simulink model "gm_ZynqBF_2tx_fpga"  (R2018b)
settings: Solver=FixedStepDiscrete  StartTime=0.0  StopTime=10.0  FixedStep=(1/420e3)/128  RelTol=1e-3
undefined symbols (not defined in the file or in its folder): a, b, c
libraries: hdlsllib x873, simulink x349
(part 4 of 40)

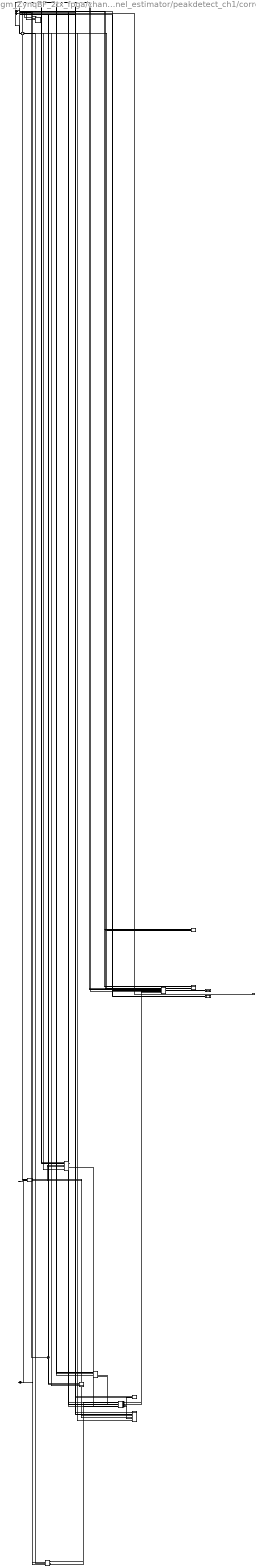
== system gm_ZynqBF_2tx_fpga/channel_estimator/peakdetect_ch1/correlator1 ==
  rx : Inport  OutDataTypeStr=fixdt(1, 16, 15)  PortDimensions=[2]  SampleTime=1.86011904761905e-08
  valid : Inport  Port=2  OutDataTypeStr=boolean  PortDimensions=1  SampleTime=1.86011904761905e-08
  en : Inport  Port=3  OutDataTypeStr=boolean  PortDimensions=1  SampleTime=1.86011904761905e-08
  rst : Inport  Port=4  OutDataTypeStr=boolean  PortDimensions=1  SampleTime=1.86011904761905e-08
  Add : Sum  AccumDataTypeStr=fixdt(1, 36, 16)  OutDataTypeStr=fixdt(1, 32, 16)  SampleTime=1.86011904761905e-08
  Compare To Constant2 : simulink/Logic and Bit Operations/Compare To Constant  relop===  const=fi(0,0,8,0,'hex','02')  OutDataTypeStr=boolean
  Compare To Constant3 : simulink/Logic and Bit Operations/Compare To Constant  relop===  const=fi(0,0,8,0,'hex','01')  OutDataTypeStr=boolean
  Constant : Constant  Value=[0;1;2;3;4;5;6;7;8;9;10;11;12;13;14;15;16;17;18;19;20;21;22;23;24;25;26;27;28;29;30;31;32;33;34;35;36;37;38;39;40;41;42;43;44;45;46;47;48;49;50;51;52;53;54;55;56;57;58;59;60;61;62;63]  OutDataTypeStr=fixdt(0, 6, 0)  SampleTime=-1
  Delay{1,4..8} (6 alike) : Delay  DelayLength=double(1)  InitialCondition=0  InputProcessing=Inherited  SampleTime=1.86011904761905e-08
  Delay2 : Delay  DelayLength=double(2)  InitialCondition=0  InputProcessing=Inherited  SampleTime=1.86011904761905e-08
  Delay3 : Delay  DelayLength=double(4)  InitialCondition=0  InputProcessing=Inherited  SampleTime=1.86011904761905e-08
  HDL Counter1 : hdlsllib/Sources/HDL Counter  CountType=Count limited  CountInit=double(0)  CountStep=double(1)  CountMax=double(2)  CountFromType=Initial value  CountFrom=double(0)  CountResetPort=off  CountLoadPort=off  CountEnbPort=on  CountDirPort=off  CountDataType=Unsigned  CountWordLen=8  CountFracLen=0  CountSampTime=1.86011904761905e-08
      settings: SourceProductBaseCode=HD
  Logical Operator : Logic  Operator=OR  Inputs=1  AllPortsSameDT=off  OutDataTypeStr=boolean  SampleTime=1.86011904761905e-08
  Logical Operator10 : Logic  AllPortsSameDT=off  OutDataTypeStr=boolean  SampleTime=1.86011904761905e-08
  Logical Operator4 : Logic  Inputs=1  AllPortsSameDT=off  OutDataTypeStr=boolean  SampleTime=1.86011904761905e-08
  Logical Operator5 : Logic  Inputs=1  AllPortsSameDT=off  OutDataTypeStr=boolean  SampleTime=1.86011904761905e-08
  Logical Operator6 : Logic  AllPortsSameDT=off  OutDataTypeStr=boolean  SampleTime=1.86011904761905e-08
  Logical Operator8 : Logic  AllPortsSameDT=off  OutDataTypeStr=boolean  SampleTime=1.86011904761905e-08
  Logical Operator9 : Logic  Operator=OR  Inputs=3  AllPortsSameDT=off  OutDataTypeStr=boolean  SampleTime=1.86011904761905e-08
  Sum of Elements1 : Sum  Inputs=+  AccumDataTypeStr=fixdt(1, 35, 16)  OutDataTypeStr=fixdt(1, 35, 16)  SampleTime=1.86011904761905e-08
  Sum of Elements2 : Sum  Inputs=+  AccumDataTypeStr=fixdt(1, 35, 16)  OutDataTypeStr=fixdt(1, 35, 16)  SampleTime=1.86011904761905e-08
  all_u : Subsystem
  all_u1 : Subsystem
  correlation_config : Subsystem
  correlator_en : Subsystem
  correlator_i_instance1 : Subsystem
  correlator_i_instance10 : Subsystem
  correlator_i_instance11 : Subsystem
  correlator_i_instance12 : Subsystem
  correlator_i_instance13 : Subsystem
  correlator_i_instance14 : Subsystem
  correlator_i_instance15 : Subsystem
  correlator_i_instance16 : Subsystem
  correlator_i_instance17 : Subsystem
  correlator_i_instance18 : Subsystem
  correlator_i_instance19 : Subsystem
  correlator_i_instance2 : Subsystem
  correlator_i_instance20 : Subsystem
  correlator_i_instance21 : Subsystem
  correlator_i_instance22 : Subsystem
  correlator_i_instance23 : Subsystem
  correlator_i_instance24 : Subsystem
  correlator_i_instance25 : Subsystem
  correlator_i_instance26 : Subsystem
  correlator_i_instance27 : Subsystem
  correlator_i_instance28 : Subsystem
  correlator_i_instance29 : Subsystem
  correlator_i_instance3 : Subsystem
  correlator_i_instance30 : Subsystem
  correlator_i_instance31 : Subsystem
  correlator_i_instance32 : Subsystem
  correlator_i_instance33 : Subsystem
  correlator_i_instance34 : Subsystem
  correlator_i_instance35 : Subsystem
  correlator_i_instance36 : Subsystem
  correlator_i_instance37 : Subsystem
  correlator_i_instance38 : Subsystem
  correlator_i_instance39 : Subsystem
  correlator_i_instance4 : Subsystem
  correlator_i_instance40 : Subsystem
  correlator_i_instance41 : Subsystem
  correlator_i_instance42 : Subsystem
  correlator_i_instance43 : Subsystem
  correlator_i_instance44 : Subsystem
  correlator_i_instance45 : Subsystem
  correlator_i_instance46 : Subsystem
  correlator_i_instance47 : Subsystem
  correlator_i_instance48 : Subsystem
  correlator_i_instance49 : Subsystem
  correlator_i_instance5 : Subsystem
  correlator_i_instance50 : Subsystem
  correlator_i_instance51 : Subsystem
  correlator_i_instance52 : Subsystem
  correlator_i_instance53 : Subsystem
  correlator_i_instance54 : Subsystem
  correlator_i_instance55 : Subsystem
  correlator_i_instance56 : Subsystem
  correlator_i_instance57 : Subsystem
  correlator_i_instance58 : Subsystem
  correlator_i_instance59 : Subsystem
  correlator_i_instance6 : Subsystem
  correlator_i_instance60 : Subsystem
  correlator_i_instance61 : Subsystem
  correlator_i_instance62 : Subsystem
  correlator_i_instance63 : Subsystem
  correlator_i_instance64 : Subsystem
  correlator_i_instance7 : Subsystem
  correlator_i_instance8 : Subsystem
  correlator_i_instance9 : Subsystem
  correlator_q_instance1 : Subsystem
  correlator_q_instance10 : Subsystem
  correlator_q_instance11 : Subsystem
  correlator_q_instance12 : Subsystem
  correlator_q_instance13 : Subsystem
  correlator_q_instance14 : Subsystem
  correlator_q_instance15 : Subsystem
  correlator_q_instance16 : Subsystem
  correlator_q_instance17 : Subsystem
  correlator_q_instance18 : Subsystem
  correlator_q_instance19 : Subsystem
  correlator_q_instance2 : Subsystem
  correlator_q_instance20 : Subsystem
  correlator_q_instance21 : Subsystem
  correlator_q_instance22 : Subsystem
  correlator_q_instance23 : Subsystem
  correlator_q_instance24 : Subsystem
  correlator_q_instance25 : Subsystem
  correlator_q_instance26 : Subsystem
  correlator_q_instance27 : Subsystem
  correlator_q_instance28 : Subsystem
  correlator_q_instance29 : Subsystem
  correlator_q_instance3 : Subsystem
  correlator_q_instance30 : Subsystem
  correlator_q_instance31 : Subsystem
  correlator_q_instance32 : Subsystem
  correlator_q_instance33 : Subsystem
  correlator_q_instance34 : Subsystem
  correlator_q_instance35 : Subsystem
  correlator_q_instance36 : Subsystem
  correlator_q_instance37 : Subsystem
  correlator_q_instance38 : Subsystem
  correlator_q_instance39 : Subsystem
  correlator_q_instance4 : Subsystem
  correlator_q_instance40 : Subsystem
  correlator_q_instance41 : Subsystem
  correlator_q_instance42 : Subsystem
  correlator_q_instance43 : Subsystem
  correlator_q_instance44 : Subsystem
  correlator_q_instance45 : Subsystem
  correlator_q_instance46 : Subsystem
  correlator_q_instance47 : Subsystem
  correlator_q_instance48 : Subsystem
  correlator_q_instance49 : Subsystem
  correlator_q_instance5 : Subsystem
  correlator_q_instance50 : Subsystem
  correlator_q_instance51 : Subsystem
  correlator_q_instance52 : Subsystem
  correlator_q_instance53 : Subsystem
  correlator_q_instance54 : Subsystem
  correlator_q_instance55 : Subsystem
  correlator_q_instance56 : Subsystem
  correlator_q_instance57 : Subsystem
  correlator_q_instance58 : Subsystem
  correlator_q_instance59 : Subsystem
  correlator_q_instance6 : Subsystem
  correlator_q_instance60 : Subsystem
  correlator_q_instance61 : Subsystem
  correlator_q_instance62 : Subsystem
  correlator_q_instance63 : Subsystem
  correlator_q_instance64 : Subsystem
  correlator_q_instance7 : Subsystem
  correlator_q_instance8 : Subsystem
  correlator_q_instance9 : Subsystem
  data_in : Subsystem
  gold_sequences : Subsystem
  rx_ram_i_instance1 : Subsystem
  rx_ram_i_instance10 : Subsystem
  rx_ram_i_instance11 : Subsystem
  rx_ram_i_instance12 : Subsystem
  rx_ram_i_instance13 : Subsystem
  rx_ram_i_instance14 : Subsystem
  rx_ram_i_instance15 : Subsystem
  rx_ram_i_instance16 : Subsystem
  rx_ram_i_instance17 : Subsystem
  rx_ram_i_instance18 : Subsystem
  rx_ram_i_instance19 : Subsystem
  rx_ram_i_instance2 : Subsystem
  rx_ram_i_instance20 : Subsystem
  rx_ram_i_instance21 : Subsystem
  rx_ram_i_instance22 : Subsystem
  rx_ram_i_instance23 : Subsystem
  rx_ram_i_instance24 : Subsystem
  rx_ram_i_instance25 : Subsystem
  rx_ram_i_instance26 : Subsystem
  rx_ram_i_instance27 : Subsystem
  rx_ram_i_instance28 : Subsystem
  rx_ram_i_instance29 : Subsystem
  rx_ram_i_instance3 : Subsystem
  rx_ram_i_instance30 : Subsystem
  rx_ram_i_instance31 : Subsystem
  rx_ram_i_instance32 : Subsystem
  rx_ram_i_instance33 : Subsystem
  rx_ram_i_instance34 : Subsystem
  rx_ram_i_instance35 : Subsystem
  rx_ram_i_instance36 : Subsystem
  rx_ram_i_instance37 : Subsystem
  rx_ram_i_instance38 : Subsystem
  rx_ram_i_instance39 : Subsystem
  rx_ram_i_instance4 : Subsystem
  rx_ram_i_instance40 : Subsystem
  rx_ram_i_instance41 : Subsystem
  rx_ram_i_instance42 : Subsystem
  rx_ram_i_instance43 : Subsystem
  rx_ram_i_instance44 : Subsystem
  rx_ram_i_instance45 : Subsystem
  rx_ram_i_instance46 : Subsystem
  rx_ram_i_instance47 : Subsystem
  rx_ram_i_instance48 : Subsystem
  rx_ram_i_instance49 : Subsystem
  rx_ram_i_instance5 : Subsystem
  rx_ram_i_instance50 : Subsystem
  rx_ram_i_instance51 : Subsystem
  rx_ram_i_instance52 : Subsystem
  rx_ram_i_instance53 : Subsystem
  rx_ram_i_instance54 : Subsystem
  rx_ram_i_instance55 : Subsystem
  rx_ram_i_instance56 : Subsystem
  rx_ram_i_instance57 : Subsystem
  rx_ram_i_instance58 : Subsystem
  rx_ram_i_instance59 : Subsystem
  rx_ram_i_instance6 : Subsystem
  rx_ram_i_instance60 : Subsystem
  rx_ram_i_instance61 : Subsystem
  rx_ram_i_instance62 : Subsystem
  rx_ram_i_instance63 : Subsystem
  rx_ram_i_instance64 : Subsystem
  rx_ram_i_instance7 : Subsystem
  rx_ram_i_instance8 : Subsystem
  rx_ram_i_instance9 : Subsystem
  rx_ram_q_instance1 : Subsystem
  rx_ram_q_instance10 : Subsystem
  rx_ram_q_instance11 : Subsystem
  rx_ram_q_instance12 : Subsystem
  rx_ram_q_instance13 : Subsystem
  rx_ram_q_instance14 : Subsystem
  rx_ram_q_instance15 : Subsystem
  rx_ram_q_instance16 : Subsystem
  rx_ram_q_instance17 : Subsystem
  rx_ram_q_instance18 : Subsystem
  rx_ram_q_instance19 : Subsystem
  rx_ram_q_instance2 : Subsystem
  rx_ram_q_instance20 : Subsystem
  rx_ram_q_instance21 : Subsystem
  rx_ram_q_instance22 : Subsystem
  rx_ram_q_instance23 : Subsystem
  rx_ram_q_instance24 : Subsystem
  rx_ram_q_instance25 : Subsystem
  rx_ram_q_instance26 : Subsystem
  rx_ram_q_instance27 : Subsystem
  rx_ram_q_instance28 : Subsystem
  rx_ram_q_instance29 : Subsystem
  rx_ram_q_instance3 : Subsystem
  rx_ram_q_instance30 : Subsystem
  rx_ram_q_instance31 : Subsystem
  rx_ram_q_instance32 : Subsystem
  rx_ram_q_instance33 : Subsystem
  rx_ram_q_instance34 : Subsystem
  rx_ram_q_instance35 : Subsystem
  rx_ram_q_instance36 : Subsystem
  rx_ram_q_instance37 : Subsystem
  rx_ram_q_instance38 : Subsystem
  rx_ram_q_instance39 : Subsystem
  rx_ram_q_instance4 : Subsystem
  rx_ram_q_instance40 : Subsystem
  rx_ram_q_instance41 : Subsystem
  rx_ram_q_instance42 : Subsystem
  rx_ram_q_instance43 : Subsystem
  rx_ram_q_instance44 : Subsystem
  rx_ram_q_instance45 : Subsystem
  rx_ram_q_instance46 : Subsystem
  rx_ram_q_instance47 : Subsystem
  rx_ram_q_instance48 : Subsystem
  rx_ram_q_instance49 : Subsystem
  rx_ram_q_instance5 : Subsystem
  rx_ram_q_instance50 : Subsystem
  rx_ram_q_instance51 : Subsystem
  rx_ram_q_instance52 : Subsystem
  rx_ram_q_instance53 : Subsystem
  rx_ram_q_instance54 : Subsystem
  rx_ram_q_instance55 : Subsystem
  rx_ram_q_instance56 : Subsystem
  rx_ram_q_instance57 : Subsystem
  rx_ram_q_instance58 : Subsystem
  rx_ram_q_instance59 : Subsystem
  rx_ram_q_instance6 : Subsystem
  rx_ram_q_instance60 : Subsystem
  rx_ram_q_instance61 : Subsystem
  rx_ram_q_instance62 : Subsystem
  rx_ram_q_instance63 : Subsystem
  rx_ram_q_instance64 : Subsystem
  rx_ram_q_instance7 : Subsystem
  rx_ram_q_instance8 : Subsystem
  rx_ram_q_instance9 : Subsystem
  select_rx_i : Selector  IndexMode=Zero-based  SampleTime=1.86011904761905e-08  IndexOptions=Index vector (dialog)  Indices=double(0)  OutputSizes=double(1)
  select_rx_q : Selector  IndexMode=Zero-based  SampleTime=1.86011904761905e-08  IndexOptions=Index vector (dialog)  Indices=double(1)  OutputSizes=double(1)
  shift_rx : Subsystem
  shift_rx1 : Subsystem
  sum_elements_i_instance1 : Subsystem
  sum_elements_i_instance2 : Subsystem
  sum_elements_i_instance3 : Subsystem
  sum_elements_i_instance4 : Subsystem
  sum_elements_i_instance5 : Subsystem
  sum_elements_i_instance6 : Subsystem
  sum_elements_i_instance7 : Subsystem
  sum_elements_i_instance8 : Subsystem
  sum_elements_q_instance1 : Subsystem
  sum_elements_q_instance2 : Subsystem
  sum_elements_q_instance3 : Subsystem
  sum_elements_q_instance4 : Subsystem
  sum_elements_q_instance5 : Subsystem
  sum_elements_q_instance6 : Subsystem
  sum_elements_q_instance7 : Subsystem
  sum_elements_q_instance8 : Subsystem
  t{,1,4..5,8,10} (6 alike) : Demux  Outputs=64
  t{2..3,6..7,9,11} (6 alike) : Mux  Inputs=64
  t12 : Demux  Outputs=8
  t{13..14,16..17} (4 alike) : Mux  Inputs=8
  t15 : Demux  Outputs=8
  dout : Outport
  dval : Outport  Port=2
  step : Outport  Port=3
  wires:
  rx/1 -> select_rx_q/1, select_rx_i/1
  valid/1 -> data_in/2(valid)
  en/1 -> Logical Operator10/2
  rst/1 -> correlation_config/1(rst), data_in/1(rst)
  Add/1 -> Delay7/1
  Compare To Constant2/1 -> Logical Operator9/3, step/1
  Compare To Constant3/1 -> Logical Operator10/1
  Constant/1 -> t10/1, t8/1
  Delay1/1 -> Add/1
  Delay2/1 -> sum_elements_q_instance8/2(start), sum_elements_q_instance7/2(start), sum_elements_q_instance6/2(start), sum_elements_q_instance5/2(start), sum_elements_q_instance4/2(start), sum_elements_q_instance3/2(start), sum_elements_q_instance2/2(start), sum_elements_i_instance8/2(start), sum_elements_i_instance7/2(start), sum_elements_i_instance6/2(start), sum_elements_i_instance5/2(start), sum_elements_i_instance4/2(start), sum_elements_i_instance3/2(start), sum_elements_i_instance2/2(start), sum_elements_i_instance1/2(start), sum_elements_q_instance1/2(start)
  Delay3/1 -> Logical Operator9/2, dval/1
  Delay4/1 -> Delay8/1, Delay6/1, rx_ram_q_instance64/6(shift), rx_ram_q_instance63/6(shift), rx_ram_q_instance62/6(shift), rx_ram_q_instance61/6(shift), rx_ram_q_instance60/6(shift), rx_ram_q_instance59/6(shift), rx_ram_q_instance58/6(shift), rx_ram_q_instance57/6(shift), rx_ram_q_instance56/6(shift), rx_ram_q_instance55/6(shift), rx_ram_q_instance54/6(shift), rx_ram_q_instance53/6(shift), rx_ram_q_instance52/6(shift), rx_ram_q_instance51/6(shift), rx_ram_q_instance50/6(shift), rx_ram_q_instance49/6(shift), rx_ram_q_instance48/6(shift), rx_ram_q_instance47/6(shift), rx_ram_q_instance46/6(shift), rx_ram_q_instance45/6(shift), rx_ram_q_instance44/6(shift), rx_ram_q_instance43/6(shift), rx_ram_q_instance42/6(shift), rx_ram_q_instance41/6(shift), rx_ram_q_instance40/6(shift), rx_ram_q_instance39/6(shift), rx_ram_q_instance38/6(shift), rx_ram_q_instance37/6(shift), rx_ram_q_instance36/6(shift), rx_ram_q_instance35/6(shift), rx_ram_q_instance34/6(shift), rx_ram_q_instance33/6(shift), rx_ram_q_instance32/6(shift), rx_ram_q_instance31/6(shift), rx_ram_q_instance30/6(shift), rx_ram_q_instance29/6(shift), rx_ram_q_instance28/6(shift), rx_ram_q_instance27/6(shift), rx_ram_q_instance26/6(shift), rx_ram_q_instance25/6(shift), rx_ram_q_instance24/6(shift), rx_ram_q_instance23/6(shift), rx_ram_q_instance22/6(shift), rx_ram_q_instance21/6(shift), rx_ram_q_instance20/6(shift), rx_ram_q_instance19/6(shift), rx_ram_q_instance18/6(shift), rx_ram_q_instance17/6(shift), rx_ram_q_instance16/6(shift), rx_ram_q_instance15/6(shift), rx_ram_q_instance14/6(shift), rx_ram_q_instance13/6(shift), rx_ram_q_instance12/6(shift), rx_ram_q_instance11/6(shift), rx_ram_q_instance10/6(shift), rx_ram_q_instance9/6(shift), rx_ram_q_instance8/6(shift), rx_ram_q_instance7/6(shift), rx_ram_q_instance6/6(shift), rx_ram_q_instance5/6(shift), rx_ram_q_instance4/6(shift), rx_ram_q_instance3/6(shift), rx_ram_q_instance2/6(shift), rx_ram_i_instance64/6(shift), rx_ram_i_instance63/6(shift), rx_ram_i_instance62/6(shift), rx_ram_i_instance61/6(shift), rx_ram_i_instance60/6(shift), rx_ram_i_instance59/6(shift), rx_ram_i_instance58/6(shift), rx_ram_i_instance57/6(shift), rx_ram_i_instance56/6(shift), rx_ram_i_instance55/6(shift), rx_ram_i_instance54/6(shift), rx_ram_i_instance53/6(shift), rx_ram_i_instance52/6(shift), rx_ram_i_instance51/6(shift), rx_ram_i_instance50/6(shift), rx_ram_i_instance49/6(shift), rx_ram_i_instance48/6(shift), rx_ram_i_instance47/6(shift), rx_ram_i_instance46/6(shift), rx_ram_i_instance45/6(shift), rx_ram_i_instance44/6(shift), rx_ram_i_instance43/6(shift), rx_ram_i_instance42/6(shift), rx_ram_i_instance41/6(shift), rx_ram_i_instance40/6(shift), rx_ram_i_instance39/6(shift), rx_ram_i_instance38/6(shift), rx_ram_i_instance37/6(shift), rx_ram_i_instance36/6(shift), rx_ram_i_instance35/6(shift), rx_ram_i_instance34/6(shift), rx_ram_i_instance33/6(shift), rx_ram_i_instance32/6(shift), rx_ram_i_instance31/6(shift), rx_ram_i_instance30/6(shift), rx_ram_i_instance29/6(shift), rx_ram_i_instance28/6(shift), rx_ram_i_instance27/6(shift), rx_ram_i_instance26/6(shift), rx_ram_i_instance25/6(shift), rx_ram_i_instance24/6(shift), rx_ram_i_instance23/6(shift), rx_ram_i_instance22/6(shift), rx_ram_i_instance21/6(shift), rx_ram_i_instance20/6(shift), rx_ram_i_instance19/6(shift), rx_ram_i_instance18/6(shift), rx_ram_i_instance17/6(shift), rx_ram_i_instance16/6(shift), rx_ram_i_instance15/6(shift), rx_ram_i_instance14/6(shift), rx_ram_i_instance13/6(shift), rx_ram_i_instance12/6(shift), rx_ram_i_instance11/6(shift), rx_ram_i_instance10/6(shift), rx_ram_i_instance9/6(shift), rx_ram_i_instance8/6(shift), rx_ram_i_instance7/6(shift), rx_ram_i_instance6/6(shift), rx_ram_i_instance5/6(shift), rx_ram_i_instance4/6(shift), rx_ram_i_instance3/6(shift), rx_ram_i_instance2/6(shift), rx_ram_i_instance1/6(shift), rx_ram_q_instance1/6(shift)
  Delay5/1 -> Add/2
  Delay6/1 -> shift_rx/2(shift)
  Delay7/1 -> dout/1
  Delay8/1 -> shift_rx1/2(shift)
  HDL Counter1/1 -> Compare To Constant3/1, Compare To Constant2/1
  Logical Operator/1 -> correlation_config/2(vin)
  Logical Operator10/1 -> Logical Operator9/1
  Logical Operator4/1 -> Logical Operator6/1
  Logical Operator5/1 -> Logical Operator6/2
  Logical Operator6/1 -> Delay2/1, correlator_en/2(done)
  Logical Operator8/1 -> Delay3/1
  Logical Operator9/1 -> HDL Counter1/1
  Sum of Elements1/1 -> Delay1/1
  Sum of Elements2/1 -> Delay5/1
  all_u/1(y) -> Logical Operator8/1
  all_u1/1(y) -> Logical Operator8/2
  correlation_config/1(addr) -> correlator_en/3(addri)
  correlation_config/2(shift) -> Delay4/1
  correlation_config/3(vout) -> correlator_en/1(valid)
  correlator_en/1(start) -> correlator_q_instance64/3(start), correlator_q_instance63/3(start), correlator_q_instance62/3(start), correlator_q_instance61/3(start), correlator_q_instance60/3(start), correlator_q_instance59/3(start), correlator_q_instance58/3(start), correlator_q_instance57/3(start), correlator_q_instance56/3(start), correlator_q_instance55/3(start), correlator_q_instance54/3(start), correlator_q_instance53/3(start), correlator_q_instance52/3(start), correlator_q_instance51/3(start), correlator_q_instance50/3(start), correlator_q_instance49/3(start), correlator_q_instance48/3(start), correlator_q_instance47/3(start), correlator_q_instance46/3(start), correlator_q_instance45/3(start), correlator_q_instance44/3(start), correlator_q_instance43/3(start), correlator_q_instance42/3(start), correlator_q_instance41/3(start), correlator_q_instance40/3(start), correlator_q_instance39/3(start), correlator_q_instance38/3(start), correlator_q_instance37/3(start), correlator_q_instance36/3(start), correlator_q_instance35/3(start), correlator_q_instance34/3(start), correlator_q_instance33/3(start), correlator_q_instance32/3(start), correlator_q_instance31/3(start), correlator_q_instance30/3(start), correlator_q_instance29/3(start), correlator_q_instance28/3(start), correlator_q_instance27/3(start), correlator_q_instance26/3(start), correlator_q_instance25/3(start), correlator_q_instance24/3(start), correlator_q_instance23/3(start), correlator_q_instance22/3(start), correlator_q_instance21/3(start), correlator_q_instance20/3(start), correlator_q_instance19/3(start), correlator_q_instance18/3(start), correlator_q_instance17/3(start), correlator_q_instance16/3(start), correlator_q_instance15/3(start), correlator_q_instance14/3(start), correlator_q_instance13/3(start), correlator_q_instance12/3(start), correlator_q_instance11/3(start), correlator_q_instance10/3(start), correlator_q_instance9/3(start), correlator_q_instance8/3(start), correlator_q_instance7/3(start), correlator_q_instance6/3(start), correlator_q_instance5/3(start), correlator_q_instance4/3(start), correlator_q_instance3/3(start), correlator_q_instance2/3(start), correlator_i_instance64/3(start), correlator_i_instance63/3(start), correlator_i_instance62/3(start), correlator_i_instance61/3(start), correlator_i_instance60/3(start), correlator_i_instance59/3(start), correlator_i_instance58/3(start), correlator_i_instance57/3(start), correlator_i_instance56/3(start), correlator_i_instance55/3(start), correlator_i_instance54/3(start), correlator_i_instance53/3(start), correlator_i_instance52/3(start), correlator_i_instance51/3(start), correlator_i_instance50/3(start), correlator_i_instance49/3(start), correlator_i_instance48/3(start), correlator_i_instance47/3(start), correlator_i_instance46/3(start), correlator_i_instance45/3(start), correlator_i_instance44/3(start), correlator_i_instance43/3(start), correlator_i_instance42/3(start), correlator_i_instance41/3(start), correlator_i_instance40/3(start), correlator_i_instance39/3(start), correlator_i_instance38/3(start), correlator_i_instance37/3(start), correlator_i_instance36/3(start), correlator_i_instance35/3(start), correlator_i_instance34/3(start), correlator_i_instance33/3(start), correlator_i_instance32/3(start), correlator_i_instance31/3(start), correlator_i_instance30/3(start), correlator_i_instance29/3(start), correlator_i_instance28/3(start), correlator_i_instance27/3(start), correlator_i_instance26/3(start), correlator_i_instance25/3(start), correlator_i_instance24/3(start), correlator_i_instance23/3(start), correlator_i_instance22/3(start), correlator_i_instance21/3(start), correlator_i_instance20/3(start), correlator_i_instance19/3(start), correlator_i_instance18/3(start), correlator_i_instance17/3(start), correlator_i_instance16/3(start), correlator_i_instance15/3(start), correlator_i_instance14/3(start), correlator_i_instance13/3(start), correlator_i_instance12/3(start), correlator_i_instance11/3(start), correlator_i_instance10/3(start), correlator_i_instance9/3(start), correlator_i_instance8/3(start), correlator_i_instance7/3(start), correlator_i_instance6/3(start), correlator_i_instance5/3(start), correlator_i_instance4/3(start), correlator_i_instance3/3(start), correlator_i_instance2/3(start), correlator_q_instance1/3(start), correlator_i_instance1/3(start)
  correlator_en/2(en) -> correlator_q_instance64/4(vin), correlator_q_instance63/4(vin), correlator_q_instance62/4(vin), correlator_q_instance61/4(vin), correlator_q_instance60/4(vin), correlator_q_instance59/4(vin), correlator_q_instance58/4(vin), correlator_q_instance57/4(vin), correlator_q_instance56/4(vin), correlator_q_instance55/4(vin), correlator_q_instance54/4(vin), correlator_q_instance53/4(vin), correlator_q_instance52/4(vin), correlator_q_instance51/4(vin), correlator_q_instance50/4(vin), correlator_q_instance49/4(vin), correlator_q_instance48/4(vin), correlator_q_instance47/4(vin), correlator_q_instance46/4(vin), correlator_q_instance45/4(vin), correlator_q_instance44/4(vin), correlator_q_instance43/4(vin), correlator_q_instance42/4(vin), correlator_q_instance41/4(vin), correlator_q_instance40/4(vin), correlator_q_instance39/4(vin), correlator_q_instance38/4(vin), correlator_q_instance37/4(vin), correlator_q_instance36/4(vin), correlator_q_instance35/4(vin), correlator_q_instance34/4(vin), correlator_q_instance33/4(vin), correlator_q_instance32/4(vin), correlator_q_instance31/4(vin), correlator_q_instance30/4(vin), correlator_q_instance29/4(vin), correlator_q_instance28/4(vin), correlator_q_instance27/4(vin), correlator_q_instance26/4(vin), correlator_q_instance25/4(vin), correlator_q_instance24/4(vin), correlator_q_instance23/4(vin), correlator_q_instance22/4(vin), correlator_q_instance21/4(vin), correlator_q_instance20/4(vin), correlator_q_instance19/4(vin), correlator_q_instance18/4(vin), correlator_q_instance17/4(vin), correlator_q_instance16/4(vin), correlator_q_instance15/4(vin), correlator_q_instance14/4(vin), correlator_q_instance13/4(vin), correlator_q_instance12/4(vin), correlator_q_instance11/4(vin), correlator_q_instance10/4(vin), correlator_q_instance9/4(vin), correlator_q_instance8/4(vin), correlator_q_instance7/4(vin), correlator_q_instance6/4(vin), correlator_q_instance5/4(vin), correlator_q_instance4/4(vin), correlator_q_instance3/4(vin), correlator_q_instance2/4(vin), correlator_i_instance64/4(vin), correlator_i_instance63/4(vin), correlator_i_instance62/4(vin), correlator_i_instance61/4(vin), correlator_i_instance60/4(vin), correlator_i_instance59/4(vin), correlator_i_instance58/4(vin), correlator_i_instance57/4(vin), correlator_i_instance56/4(vin), correlator_i_instance55/4(vin), correlator_i_instance54/4(vin), correlator_i_instance53/4(vin), correlator_i_instance52/4(vin), correlator_i_instance51/4(vin), correlator_i_instance50/4(vin), correlator_i_instance49/4(vin), correlator_i_instance48/4(vin), correlator_i_instance47/4(vin), correlator_i_instance46/4(vin), correlator_i_instance45/4(vin), correlator_i_instance44/4(vin), correlator_i_instance43/4(vin), correlator_i_instance42/4(vin), correlator_i_instance41/4(vin), correlator_i_instance40/4(vin), correlator_i_instance39/4(vin), correlator_i_instance38/4(vin), correlator_i_instance37/4(vin), correlator_i_instance36/4(vin), correlator_i_instance35/4(vin), correlator_i_instance34/4(vin), correlator_i_instance33/4(vin), correlator_i_instance32/4(vin), correlator_i_instance31/4(vin), correlator_i_instance30/4(vin), correlator_i_instance29/4(vin), correlator_i_instance28/4(vin), correlator_i_instance27/4(vin), correlator_i_instance26/4(vin), correlator_i_instance25/4(vin), correlator_i_instance24/4(vin), correlator_i_instance23/4(vin), correlator_i_instance22/4(vin), correlator_i_instance21/4(vin), correlator_i_instance20/4(vin), correlator_i_instance19/4(vin), correlator_i_instance18/4(vin), correlator_i_instance17/4(vin), correlator_i_instance16/4(vin), correlator_i_instance15/4(vin), correlator_i_instance14/4(vin), correlator_i_instance13/4(vin), correlator_i_instance12/4(vin), correlator_i_instance11/4(vin), correlator_i_instance10/4(vin), correlator_i_instance9/4(vin), correlator_i_instance8/4(vin), correlator_i_instance7/4(vin), correlator_i_instance6/4(vin), correlator_i_instance5/4(vin), correlator_i_instance4/4(vin), correlator_i_instance3/4(vin), correlator_i_instance2/4(vin), correlator_q_instance1/4(vin), correlator_i_instance1/4(vin)
  correlator_en/3(gs_addr) -> gold_sequences/1(addr)
  correlator_en/4(rx_addr) -> rx_ram_q_instance64/5(raddr), rx_ram_q_instance63/5(raddr), rx_ram_q_instance62/5(raddr), rx_ram_q_instance61/5(raddr), rx_ram_q_instance60/5(raddr), rx_ram_q_instance59/5(raddr), rx_ram_q_instance58/5(raddr), rx_ram_q_instance57/5(raddr), rx_ram_q_instance56/5(raddr), rx_ram_q_instance55/5(raddr), rx_ram_q_instance54/5(raddr), rx_ram_q_instance53/5(raddr), rx_ram_q_instance52/5(raddr), rx_ram_q_instance51/5(raddr), rx_ram_q_instance50/5(raddr), rx_ram_q_instance49/5(raddr), rx_ram_q_instance48/5(raddr), rx_ram_q_instance47/5(raddr), rx_ram_q_instance46/5(raddr), rx_ram_q_instance45/5(raddr), rx_ram_q_instance44/5(raddr), rx_ram_q_instance43/5(raddr), rx_ram_q_instance42/5(raddr), rx_ram_q_instance41/5(raddr), rx_ram_q_instance40/5(raddr), rx_ram_q_instance39/5(raddr), rx_ram_q_instance38/5(raddr), rx_ram_q_instance37/5(raddr), rx_ram_q_instance36/5(raddr), rx_ram_q_instance35/5(raddr), rx_ram_q_instance34/5(raddr), rx_ram_q_instance33/5(raddr), rx_ram_q_instance32/5(raddr), rx_ram_q_instance31/5(raddr), rx_ram_q_instance30/5(raddr), rx_ram_q_instance29/5(raddr), rx_ram_q_instance28/5(raddr), rx_ram_q_instance27/5(raddr), rx_ram_q_instance26/5(raddr), rx_ram_q_instance25/5(raddr), rx_ram_q_instance24/5(raddr), rx_ram_q_instance23/5(raddr), rx_ram_q_instance22/5(raddr), rx_ram_q_instance21/5(raddr), rx_ram_q_instance20/5(raddr), rx_ram_q_instance19/5(raddr), rx_ram_q_instance18/5(raddr), rx_ram_q_instance17/5(raddr), rx_ram_q_instance16/5(raddr), rx_ram_q_instance15/5(raddr), rx_ram_q_instance14/5(raddr), rx_ram_q_instance13/5(raddr), rx_ram_q_instance12/5(raddr), rx_ram_q_instance11/5(raddr), rx_ram_q_instance10/5(raddr), rx_ram_q_instance9/5(raddr), rx_ram_q_instance8/5(raddr), rx_ram_q_instance7/5(raddr), rx_ram_q_instance6/5(raddr), rx_ram_q_instance5/5(raddr), rx_ram_q_instance4/5(raddr), rx_ram_q_instance3/5(raddr), rx_ram_q_instance2/5(raddr), rx_ram_i_instance64/5(raddr), rx_ram_i_instance63/5(raddr), rx_ram_i_instance62/5(raddr), rx_ram_i_instance61/5(raddr), rx_ram_i_instance60/5(raddr), rx_ram_i_instance59/5(raddr), rx_ram_i_instance58/5(raddr), rx_ram_i_instance57/5(raddr), rx_ram_i_instance56/5(raddr), rx_ram_i_instance55/5(raddr), rx_ram_i_instance54/5(raddr), rx_ram_i_instance53/5(raddr), rx_ram_i_instance52/5(raddr), rx_ram_i_instance51/5(raddr), rx_ram_i_instance50/5(raddr), rx_ram_i_instance49/5(raddr), rx_ram_i_instance48/5(raddr), rx_ram_i_instance47/5(raddr), rx_ram_i_instance46/5(raddr), rx_ram_i_instance45/5(raddr), rx_ram_i_instance44/5(raddr), rx_ram_i_instance43/5(raddr), rx_ram_i_instance42/5(raddr), rx_ram_i_instance41/5(raddr), rx_ram_i_instance40/5(raddr), rx_ram_i_instance39/5(raddr), rx_ram_i_instance38/5(raddr), rx_ram_i_instance37/5(raddr), rx_ram_i_instance36/5(raddr), rx_ram_i_instance35/5(raddr), rx_ram_i_instance34/5(raddr), rx_ram_i_instance33/5(raddr), rx_ram_i_instance32/5(raddr), rx_ram_i_instance31/5(raddr), rx_ram_i_instance30/5(raddr), rx_ram_i_instance29/5(raddr), rx_ram_i_instance28/5(raddr), rx_ram_i_instance27/5(raddr), rx_ram_i_instance26/5(raddr), rx_ram_i_instance25/5(raddr), rx_ram_i_instance24/5(raddr), rx_ram_i_instance23/5(raddr), rx_ram_i_instance22/5(raddr), rx_ram_i_instance21/5(raddr), rx_ram_i_instance20/5(raddr), rx_ram_i_instance19/5(raddr), rx_ram_i_instance18/5(raddr), rx_ram_i_instance17/5(raddr), rx_ram_i_instance16/5(raddr), rx_ram_i_instance15/5(raddr), rx_ram_i_instance14/5(raddr), rx_ram_i_instance13/5(raddr), rx_ram_i_instance12/5(raddr), rx_ram_i_instance11/5(raddr), rx_ram_i_instance10/5(raddr), rx_ram_i_instance9/5(raddr), rx_ram_i_instance8/5(raddr), rx_ram_i_instance7/5(raddr), rx_ram_i_instance6/5(raddr), rx_ram_i_instance5/5(raddr), rx_ram_i_instance4/5(raddr), rx_ram_i_instance3/5(raddr), rx_ram_i_instance2/5(raddr), rx_ram_i_instance1/5(raddr), rx_ram_q_instance1/5(raddr)
  t2/1 -> t12/1
  t3/1 -> Logical Operator4/1
  t6/1 -> t15/1
  t7/1 -> Logical Operator5/1
  data_in/1(addr) -> rx_ram_q_instance64/3(waddr), rx_ram_q_instance63/3(waddr), rx_ram_q_instance62/3(waddr), rx_ram_q_instance61/3(waddr), rx_ram_q_instance60/3(waddr), rx_ram_q_instance59/3(waddr), rx_ram_q_instance58/3(waddr), rx_ram_q_instance57/3(waddr), rx_ram_q_instance56/3(waddr), rx_ram_q_instance55/3(waddr), rx_ram_q_instance54/3(waddr), rx_ram_q_instance53/3(waddr), rx_ram_q_instance52/3(waddr), rx_ram_q_instance51/3(waddr), rx_ram_q_instance50/3(waddr), rx_ram_q_instance49/3(waddr), rx_ram_q_instance48/3(waddr), rx_ram_q_instance47/3(waddr), rx_ram_q_instance46/3(waddr), rx_ram_q_instance45/3(waddr), rx_ram_q_instance44/3(waddr), rx_ram_q_instance43/3(waddr), rx_ram_q_instance42/3(waddr), rx_ram_q_instance41/3(waddr), rx_ram_q_instance40/3(waddr), rx_ram_q_instance39/3(waddr), rx_ram_q_instance38/3(waddr), rx_ram_q_instance37/3(waddr), rx_ram_q_instance36/3(waddr), rx_ram_q_instance35/3(waddr), rx_ram_q_instance34/3(waddr), rx_ram_q_instance33/3(waddr), rx_ram_q_instance32/3(waddr), rx_ram_q_instance31/3(waddr), rx_ram_q_instance30/3(waddr), rx_ram_q_instance29/3(waddr), rx_ram_q_instance28/3(waddr), rx_ram_q_instance27/3(waddr), rx_ram_q_instance26/3(waddr), rx_ram_q_instance25/3(waddr), rx_ram_q_instance24/3(waddr), rx_ram_q_instance23/3(waddr), rx_ram_q_instance22/3(waddr), rx_ram_q_instance21/3(waddr), rx_ram_q_instance20/3(waddr), rx_ram_q_instance19/3(waddr), rx_ram_q_instance18/3(waddr), rx_ram_q_instance17/3(waddr), rx_ram_q_instance16/3(waddr), rx_ram_q_instance15/3(waddr), rx_ram_q_instance14/3(waddr), rx_ram_q_instance13/3(waddr), rx_ram_q_instance12/3(waddr), rx_ram_q_instance11/3(waddr), rx_ram_q_instance10/3(waddr), rx_ram_q_instance9/3(waddr), rx_ram_q_instance8/3(waddr), rx_ram_q_instance7/3(waddr), rx_ram_q_instance6/3(waddr), rx_ram_q_instance5/3(waddr), rx_ram_q_instance4/3(waddr), rx_ram_q_instance3/3(waddr), rx_ram_q_instance2/3(waddr), rx_ram_i_instance64/3(waddr), rx_ram_i_instance63/3(waddr), rx_ram_i_instance62/3(waddr), rx_ram_i_instance61/3(waddr), rx_ram_i_instance60/3(waddr), rx_ram_i_instance59/3(waddr), rx_ram_i_instance58/3(waddr), rx_ram_i_instance57/3(waddr), rx_ram_i_instance56/3(waddr), rx_ram_i_instance55/3(waddr), rx_ram_i_instance54/3(waddr), rx_ram_i_instance53/3(waddr), rx_ram_i_instance52/3(waddr), rx_ram_i_instance51/3(waddr), rx_ram_i_instance50/3(waddr), rx_ram_i_instance49/3(waddr), rx_ram_i_instance48/3(waddr), rx_ram_i_instance47/3(waddr), rx_ram_i_instance46/3(waddr), rx_ram_i_instance45/3(waddr), rx_ram_i_instance44/3(waddr), rx_ram_i_instance43/3(waddr), rx_ram_i_instance42/3(waddr), rx_ram_i_instance41/3(waddr), rx_ram_i_instance40/3(waddr), rx_ram_i_instance39/3(waddr), rx_ram_i_instance38/3(waddr), rx_ram_i_instance37/3(waddr), rx_ram_i_instance36/3(waddr), rx_ram_i_instance35/3(waddr), rx_ram_i_instance34/3(waddr), rx_ram_i_instance33/3(waddr), rx_ram_i_instance32/3(waddr), rx_ram_i_instance31/3(waddr), rx_ram_i_instance30/3(waddr), rx_ram_i_instance29/3(waddr), rx_ram_i_instance28/3(waddr), rx_ram_i_instance27/3(waddr), rx_ram_i_instance26/3(waddr), rx_ram_i_instance25/3(waddr), rx_ram_i_instance24/3(waddr), rx_ram_i_instance23/3(waddr), rx_ram_i_instance22/3(waddr), rx_ram_i_instance21/3(waddr), rx_ram_i_instance20/3(waddr), rx_ram_i_instance19/3(waddr), rx_ram_i_instance18/3(waddr), rx_ram_i_instance17/3(waddr), rx_ram_i_instance16/3(waddr), rx_ram_i_instance15/3(waddr), rx_ram_i_instance14/3(waddr), rx_ram_i_instance13/3(waddr), rx_ram_i_instance12/3(waddr), rx_ram_i_instance11/3(waddr), rx_ram_i_instance10/3(waddr), rx_ram_i_instance9/3(waddr), rx_ram_i_instance8/3(waddr), rx_ram_i_instance7/3(waddr), rx_ram_i_instance6/3(waddr), rx_ram_i_instance5/3(waddr), rx_ram_i_instance4/3(waddr), rx_ram_i_instance3/3(waddr), rx_ram_i_instance2/3(waddr), rx_ram_q_instance1/3(waddr), rx_ram_i_instance1/3(waddr)
  data_in/2(we) -> Logical Operator/1, rx_ram_q_instance64/4(we), rx_ram_q_instance63/4(we), rx_ram_q_instance62/4(we), rx_ram_q_instance61/4(we), rx_ram_q_instance60/4(we), rx_ram_q_instance59/4(we), rx_ram_q_instance58/4(we), rx_ram_q_instance57/4(we), rx_ram_q_instance56/4(we), rx_ram_q_instance55/4(we), rx_ram_q_instance54/4(we), rx_ram_q_instance53/4(we), rx_ram_q_instance52/4(we), rx_ram_q_instance51/4(we), rx_ram_q_instance50/4(we), rx_ram_q_instance49/4(we), rx_ram_q_instance48/4(we), rx_ram_q_instance47/4(we), rx_ram_q_instance46/4(we), rx_ram_q_instance45/4(we), rx_ram_q_instance44/4(we), rx_ram_q_instance43/4(we), rx_ram_q_instance42/4(we), rx_ram_q_instance41/4(we), rx_ram_q_instance40/4(we), rx_ram_q_instance39/4(we), rx_ram_q_instance38/4(we), rx_ram_q_instance37/4(we), rx_ram_q_instance36/4(we), rx_ram_q_instance35/4(we), rx_ram_q_instance34/4(we), rx_ram_q_instance33/4(we), rx_ram_q_instance32/4(we), rx_ram_q_instance31/4(we), rx_ram_q_instance30/4(we), rx_ram_q_instance29/4(we), rx_ram_q_instance28/4(we), rx_ram_q_instance27/4(we), rx_ram_q_instance26/4(we), rx_ram_q_instance25/4(we), rx_ram_q_instance24/4(we), rx_ram_q_instance23/4(we), rx_ram_q_instance22/4(we), rx_ram_q_instance21/4(we), rx_ram_q_instance20/4(we), rx_ram_q_instance19/4(we), rx_ram_q_instance18/4(we), rx_ram_q_instance17/4(we), rx_ram_q_instance16/4(we), rx_ram_q_instance15/4(we), rx_ram_q_instance14/4(we), rx_ram_q_instance13/4(we), rx_ram_q_instance12/4(we), rx_ram_q_instance11/4(we), rx_ram_q_instance10/4(we), rx_ram_q_instance9/4(we), rx_ram_q_instance8/4(we), rx_ram_q_instance7/4(we), rx_ram_q_instance6/4(we), rx_ram_q_instance5/4(we), rx_ram_q_instance4/4(we), rx_ram_q_instance3/4(we), rx_ram_q_instance2/4(we), rx_ram_i_instance64/4(we), rx_ram_i_instance63/4(we), rx_ram_i_instance62/4(we), rx_ram_i_instance61/4(we), rx_ram_i_instance60/4(we), rx_ram_i_instance59/4(we), rx_ram_i_instance58/4(we), rx_ram_i_instance57/4(we), rx_ram_i_instance56/4(we), rx_ram_i_instance55/4(we), rx_ram_i_instance54/4(we), rx_ram_i_instance53/4(we), rx_ram_i_instance52/4(we), rx_ram_i_instance51/4(we), rx_ram_i_instance50/4(we), rx_ram_i_instance49/4(we), rx_ram_i_instance48/4(we), rx_ram_i_instance47/4(we), rx_ram_i_instance46/4(we), rx_ram_i_instance45/4(we), rx_ram_i_instance44/4(we), rx_ram_i_instance43/4(we), rx_ram_i_instance42/4(we), rx_ram_i_instance41/4(we), rx_ram_i_instance40/4(we), rx_ram_i_instance39/4(we), rx_ram_i_instance38/4(we), rx_ram_i_instance37/4(we), rx_ram_i_instance36/4(we), rx_ram_i_instance35/4(we), rx_ram_i_instance34/4(we), rx_ram_i_instance33/4(we), rx_ram_i_instance32/4(we), rx_ram_i_instance31/4(we), rx_ram_i_instance30/4(we), rx_ram_i_instance29/4(we), rx_ram_i_instance28/4(we), rx_ram_i_instance27/4(we), rx_ram_i_instance26/4(we), rx_ram_i_instance25/4(we), rx_ram_i_instance24/4(we), rx_ram_i_instance23/4(we), rx_ram_i_instance22/4(we), rx_ram_i_instance21/4(we), rx_ram_i_instance20/4(we), rx_ram_i_instance19/4(we), rx_ram_i_instance18/4(we), rx_ram_i_instance17/4(we), rx_ram_i_instance16/4(we), rx_ram_i_instance15/4(we), rx_ram_i_instance14/4(we), rx_ram_i_instance13/4(we), rx_ram_i_instance12/4(we), rx_ram_i_instance11/4(we), rx_ram_i_instance10/4(we), rx_ram_i_instance9/4(we), rx_ram_i_instance8/4(we), rx_ram_i_instance7/4(we), rx_ram_i_instance6/4(we), rx_ram_i_instance5/4(we), rx_ram_i_instance4/4(we), rx_ram_i_instance3/4(we), rx_ram_i_instance2/4(we), rx_ram_q_instance1/4(we), rx_ram_i_instance1/4(we)
  gold_sequences/1(gs1_i) -> t1/1
  gold_sequences/2(gs1_q) -> t5/1
  t9/1 -> shift_rx/1(u)
  t11/1 -> shift_rx1/1(u)
  select_rx_i/1 -> rx_ram_i_instance64/2(wdata), rx_ram_i_instance63/2(wdata), rx_ram_i_instance62/2(wdata), rx_ram_i_instance61/2(wdata), rx_ram_i_instance60/2(wdata), rx_ram_i_instance59/2(wdata), rx_ram_i_instance58/2(wdata), rx_ram_i_instance57/2(wdata), rx_ram_i_instance56/2(wdata), rx_ram_i_instance55/2(wdata), rx_ram_i_instance54/2(wdata), rx_ram_i_instance53/2(wdata), rx_ram_i_instance52/2(wdata), rx_ram_i_instance51/2(wdata), rx_ram_i_instance50/2(wdata), rx_ram_i_instance49/2(wdata), rx_ram_i_instance48/2(wdata), rx_ram_i_instance47/2(wdata), rx_ram_i_instance46/2(wdata), rx_ram_i_instance45/2(wdata), rx_ram_i_instance44/2(wdata), rx_ram_i_instance43/2(wdata), rx_ram_i_instance42/2(wdata), rx_ram_i_instance41/2(wdata), rx_ram_i_instance40/2(wdata), rx_ram_i_instance39/2(wdata), rx_ram_i_instance38/2(wdata), rx_ram_i_instance37/2(wdata), rx_ram_i_instance36/2(wdata), rx_ram_i_instance35/2(wdata), rx_ram_i_instance34/2(wdata), rx_ram_i_instance33/2(wdata), rx_ram_i_instance32/2(wdata), rx_ram_i_instance31/2(wdata), rx_ram_i_instance30/2(wdata), rx_ram_i_instance29/2(wdata), rx_ram_i_instance28/2(wdata), rx_ram_i_instance27/2(wdata), rx_ram_i_instance26/2(wdata), rx_ram_i_instance25/2(wdata), rx_ram_i_instance24/2(wdata), rx_ram_i_instance23/2(wdata), rx_ram_i_instance22/2(wdata), rx_ram_i_instance21/2(wdata), rx_ram_i_instance20/2(wdata), rx_ram_i_instance19/2(wdata), rx_ram_i_instance18/2(wdata), rx_ram_i_instance17/2(wdata), rx_ram_i_instance16/2(wdata), rx_ram_i_instance15/2(wdata), rx_ram_i_instance14/2(wdata), rx_ram_i_instance13/2(wdata), rx_ram_i_instance12/2(wdata), rx_ram_i_instance11/2(wdata), rx_ram_i_instance10/2(wdata), rx_ram_i_instance9/2(wdata), rx_ram_i_instance8/2(wdata), rx_ram_i_instance7/2(wdata), rx_ram_i_instance6/2(wdata), rx_ram_i_instance5/2(wdata), rx_ram_i_instance4/2(wdata), rx_ram_i_instance3/2(wdata), rx_ram_i_instance2/2(wdata), rx_ram_i_instance1/2(wdata)
  select_rx_q/1 -> rx_ram_q_instance64/2(wdata), rx_ram_q_instance63/2(wdata), rx_ram_q_instance62/2(wdata), rx_ram_q_instance61/2(wdata), rx_ram_q_instance60/2(wdata), rx_ram_q_instance59/2(wdata), rx_ram_q_instance58/2(wdata), rx_ram_q_instance57/2(wdata), rx_ram_q_instance56/2(wdata), rx_ram_q_instance55/2(wdata), rx_ram_q_instance54/2(wdata), rx_ram_q_instance53/2(wdata), rx_ram_q_instance52/2(wdata), rx_ram_q_instance51/2(wdata), rx_ram_q_instance50/2(wdata), rx_ram_q_instance49/2(wdata), rx_ram_q_instance48/2(wdata), rx_ram_q_instance47/2(wdata), rx_ram_q_instance46/2(wdata), rx_ram_q_instance45/2(wdata), rx_ram_q_instance44/2(wdata), rx_ram_q_instance43/2(wdata), rx_ram_q_instance42/2(wdata), rx_ram_q_instance41/2(wdata), rx_ram_q_instance40/2(wdata), rx_ram_q_instance39/2(wdata), rx_ram_q_instance38/2(wdata), rx_ram_q_instance37/2(wdata), rx_ram_q_instance36/2(wdata), rx_ram_q_instance35/2(wdata), rx_ram_q_instance34/2(wdata), rx_ram_q_instance33/2(wdata), rx_ram_q_instance32/2(wdata), rx_ram_q_instance31/2(wdata), rx_ram_q_instance30/2(wdata), rx_ram_q_instance29/2(wdata), rx_ram_q_instance28/2(wdata), rx_ram_q_instance27/2(wdata), rx_ram_q_instance26/2(wdata), rx_ram_q_instance25/2(wdata), rx_ram_q_instance24/2(wdata), rx_ram_q_instance23/2(wdata), rx_ram_q_instance22/2(wdata), rx_ram_q_instance21/2(wdata), rx_ram_q_instance20/2(wdata), rx_ram_q_instance19/2(wdata), rx_ram_q_instance18/2(wdata), rx_ram_q_instance17/2(wdata), rx_ram_q_instance16/2(wdata), rx_ram_q_instance15/2(wdata), rx_ram_q_instance14/2(wdata), rx_ram_q_instance13/2(wdata), rx_ram_q_instance12/2(wdata), rx_ram_q_instance11/2(wdata), rx_ram_q_instance10/2(wdata), rx_ram_q_instance9/2(wdata), rx_ram_q_instance8/2(wdata), rx_ram_q_instance7/2(wdata), rx_ram_q_instance6/2(wdata), rx_ram_q_instance5/2(wdata), rx_ram_q_instance4/2(wdata), rx_ram_q_instance3/2(wdata), rx_ram_q_instance2/2(wdata), rx_ram_q_instance1/2(wdata)
  shift_rx/1(y) -> t/1
  shift_rx1/1(y) -> t4/1
  t13/1 -> Sum of Elements1/1
  t14/1 -> all_u/1(u)
  t16/1 -> Sum of Elements2/1
  t17/1 -> all_u1/1(u)
  t/1 -> correlator_i_instance1/1(rx)
  t/2 -> correlator_i_instance2/1(rx)
  t/3 -> correlator_i_instance3/1(rx)
  t/4 -> correlator_i_instance4/1(rx)
  t/5 -> correlator_i_instance5/1(rx)
  t/6 -> correlator_i_instance6/1(rx)
  t/7 -> correlator_i_instance7/1(rx)
  t/8 -> correlator_i_instance8/1(rx)
  t/9 -> correlator_i_instance9/1(rx)
  t/10 -> correlator_i_instance10/1(rx)
  t/11 -> correlator_i_instance11/1(rx)
  t/12 -> correlator_i_instance12/1(rx)
  t/13 -> correlator_i_instance13/1(rx)
  t/14 -> correlator_i_instance14/1(rx)
  t/15 -> correlator_i_instance15/1(rx)
  t/16 -> correlator_i_instance16/1(rx)
  t/17 -> correlator_i_instance17/1(rx)
  t/18 -> correlator_i_instance18/1(rx)
  t/19 -> correlator_i_instance19/1(rx)
  t/20 -> correlator_i_instance20/1(rx)
  t/21 -> correlator_i_instance21/1(rx)
  t/22 -> correlator_i_instance22/1(rx)
  t/23 -> correlator_i_instance23/1(rx)
  t/24 -> correlator_i_instance24/1(rx)
  t/25 -> correlator_i_instance25/1(rx)
  t/26 -> correlator_i_instance26/1(rx)
  t/27 -> correlator_i_instance27/1(rx)
  t/28 -> correlator_i_instance28/1(rx)
  t/29 -> correlator_i_instance29/1(rx)
  t/30 -> correlator_i_instance30/1(rx)
  t/31 -> correlator_i_instance31/1(rx)
  t/32 -> correlator_i_instance32/1(rx)
  t/33 -> correlator_i_instance33/1(rx)
  t/34 -> correlator_i_instance34/1(rx)
  t/35 -> correlator_i_instance35/1(rx)
  t/36 -> correlator_i_instance36/1(rx)
  t/37 -> correlator_i_instance37/1(rx)
  t/38 -> correlator_i_instance38/1(rx)
  t/39 -> correlator_i_instance39/1(rx)
  t/40 -> correlator_i_instance40/1(rx)
  t/41 -> correlator_i_instance41/1(rx)
  t/42 -> correlator_i_instance42/1(rx)
  t/43 -> correlator_i_instance43/1(rx)
  t/44 -> correlator_i_instance44/1(rx)
  t/45 -> correlator_i_instance45/1(rx)
  t/46 -> correlator_i_instance46/1(rx)
  t/47 -> correlator_i_instance47/1(rx)
  t/48 -> correlator_i_instance48/1(rx)
  t/49 -> correlator_i_instance49/1(rx)
  t/50 -> correlator_i_instance50/1(rx)
  t/51 -> correlator_i_instance51/1(rx)
  t/52 -> correlator_i_instance52/1(rx)
  t/53 -> correlator_i_instance53/1(rx)
  t/54 -> correlator_i_instance54/1(rx)
  t/55 -> correlator_i_instance55/1(rx)
  t/56 -> correlator_i_instance56/1(rx)
  t/57 -> correlator_i_instance57/1(rx)
  t/58 -> correlator_i_instance58/1(rx)
  t/59 -> correlator_i_instance59/1(rx)
  t/60 -> correlator_i_instance60/1(rx)
  t/61 -> correlator_i_instance61/1(rx)
  t/62 -> correlator_i_instance62/1(rx)
  t/63 -> correlator_i_instance63/1(rx)
  t/64 -> correlator_i_instance64/1(rx)
  t1/1 -> correlator_i_instance1/2(gs)
  t1/2 -> correlator_i_instance2/2(gs)
  t1/3 -> correlator_i_instance3/2(gs)
  t1/4 -> correlator_i_instance4/2(gs)
  t1/5 -> correlator_i_instance5/2(gs)
  t1/6 -> correlator_i_instance6/2(gs)
  t1/7 -> correlator_i_instance7/2(gs)
  t1/8 -> correlator_i_instance8/2(gs)
  t1/9 -> correlator_i_instance9/2(gs)
  t1/10 -> correlator_i_instance10/2(gs)
  t1/11 -> correlator_i_instance11/2(gs)
  t1/12 -> correlator_i_instance12/2(gs)
  t1/13 -> correlator_i_instance13/2(gs)
  t1/14 -> correlator_i_instance14/2(gs)
  t1/15 -> correlator_i_instance15/2(gs)
  t1/16 -> correlator_i_instance16/2(gs)
  t1/17 -> correlator_i_instance17/2(gs)
  t1/18 -> correlator_i_instance18/2(gs)
  t1/19 -> correlator_i_instance19/2(gs)
  t1/20 -> correlator_i_instance20/2(gs)
  t1/21 -> correlator_i_instance21/2(gs)
  t1/22 -> correlator_i_instance22/2(gs)
  t1/23 -> correlator_i_instance23/2(gs)
  t1/24 -> correlator_i_instance24/2(gs)
  t1/25 -> correlator_i_instance25/2(gs)
  t1/26 -> correlator_i_instance26/2(gs)
  t1/27 -> correlator_i_instance27/2(gs)
  t1/28 -> correlator_i_instance28/2(gs)
  t1/29 -> correlator_i_instance29/2(gs)
  t1/30 -> correlator_i_instance30/2(gs)
  t1/31 -> correlator_i_instance31/2(gs)
  t1/32 -> correlator_i_instance32/2(gs)
  t1/33 -> correlator_i_instance33/2(gs)
  t1/34 -> correlator_i_instance34/2(gs)
  t1/35 -> correlator_i_instance35/2(gs)
  t1/36 -> correlator_i_instance36/2(gs)
  t1/37 -> correlator_i_instance37/2(gs)
  t1/38 -> correlator_i_instance38/2(gs)
  t1/39 -> correlator_i_instance39/2(gs)
  t1/40 -> correlator_i_instance40/2(gs)
  t1/41 -> correlator_i_instance41/2(gs)
  t1/42 -> correlator_i_instance42/2(gs)
  t1/43 -> correlator_i_instance43/2(gs)
  t1/44 -> correlator_i_instance44/2(gs)
  t1/45 -> correlator_i_instance45/2(gs)
  t1/46 -> correlator_i_instance46/2(gs)
  t1/47 -> correlator_i_instance47/2(gs)
  t1/48 -> correlator_i_instance48/2(gs)
  t1/49 -> correlator_i_instance49/2(gs)
  t1/50 -> correlator_i_instance50/2(gs)
  t1/51 -> correlator_i_instance51/2(gs)
  t1/52 -> correlator_i_instance52/2(gs)
  t1/53 -> correlator_i_instance53/2(gs)
  t1/54 -> correlator_i_instance54/2(gs)
  t1/55 -> correlator_i_instance55/2(gs)
  t1/56 -> correlator_i_instance56/2(gs)
  t1/57 -> correlator_i_instance57/2(gs)
  t1/58 -> correlator_i_instance58/2(gs)
  t1/59 -> correlator_i_instance59/2(gs)
  t1/60 -> correlator_i_instance60/2(gs)
  t1/61 -> correlator_i_instance61/2(gs)
  t1/62 -> correlator_i_instance62/2(gs)
  t1/63 -> correlator_i_instance63/2(gs)
  t1/64 -> correlator_i_instance64/2(gs)
  correlator_i_instance1/1(dout) -> t2/1
  correlator_i_instance2/1(dout) -> t2/2
  correlator_i_instance3/1(dout) -> t2/3
  correlator_i_instance4/1(dout) -> t2/4
  correlator_i_instance5/1(dout) -> t2/5
  correlator_i_instance6/1(dout) -> t2/6
  correlator_i_instance7/1(dout) -> t2/7
  correlator_i_instance8/1(dout) -> t2/8
  correlator_i_instance9/1(dout) -> t2/9
  correlator_i_instance10/1(dout) -> t2/10
  correlator_i_instance11/1(dout) -> t2/11
  correlator_i_instance12/1(dout) -> t2/12
  correlator_i_instance13/1(dout) -> t2/13
  correlator_i_instance14/1(dout) -> t2/14
  correlator_i_instance15/1(dout) -> t2/15
  correlator_i_instance16/1(dout) -> t2/16
  correlator_i_instance17/1(dout) -> t2/17
  correlator_i_instance18/1(dout) -> t2/18
  correlator_i_instance19/1(dout) -> t2/19
  correlator_i_instance20/1(dout) -> t2/20
  correlator_i_instance21/1(dout) -> t2/21
  correlator_i_instance22/1(dout) -> t2/22
  correlator_i_instance23/1(dout) -> t2/23
  correlator_i_instance24/1(dout) -> t2/24
  correlator_i_instance25/1(dout) -> t2/25
  correlator_i_instance26/1(dout) -> t2/26
  correlator_i_instance27/1(dout) -> t2/27
  correlator_i_instance28/1(dout) -> t2/28
  correlator_i_instance29/1(dout) -> t2/29
  correlator_i_instance30/1(dout) -> t2/30
  correlator_i_instance31/1(dout) -> t2/31
  correlator_i_instance32/1(dout) -> t2/32
  correlator_i_instance33/1(dout) -> t2/33
  correlator_i_instance34/1(dout) -> t2/34
  correlator_i_instance35/1(dout) -> t2/35
  correlator_i_instance36/1(dout) -> t2/36
  correlator_i_instance37/1(dout) -> t2/37
  correlator_i_instance38/1(dout) -> t2/38
  correlator_i_instance39/1(dout) -> t2/39
  correlator_i_instance40/1(dout) -> t2/40
  correlator_i_instance41/1(dout) -> t2/41
  correlator_i_instance42/1(dout) -> t2/42
  correlator_i_instance43/1(dout) -> t2/43
  correlator_i_instance44/1(dout) -> t2/44
  correlator_i_instance45/1(dout) -> t2/45
  correlator_i_instance46/1(dout) -> t2/46
  correlator_i_instance47/1(dout) -> t2/47
  correlator_i_instance48/1(dout) -> t2/48
  correlator_i_instance49/1(dout) -> t2/49
  correlator_i_instance50/1(dout) -> t2/50
  correlator_i_instance51/1(dout) -> t2/51
  correlator_i_instance52/1(dout) -> t2/52
  correlator_i_instance53/1(dout) -> t2/53
  correlator_i_instance54/1(dout) -> t2/54
  correlator_i_instance55/1(dout) -> t2/55
  correlator_i_instance56/1(dout) -> t2/56
  correlator_i_instance57/1(dout) -> t2/57
  correlator_i_instance58/1(dout) -> t2/58
  correlator_i_instance59/1(dout) -> t2/59
  correlator_i_instance60/1(dout) -> t2/60
  correlator_i_instance61/1(dout) -> t2/61
  correlator_i_instance62/1(dout) -> t2/62
  correlator_i_instance63/1(dout) -> t2/63
  correlator_i_instance64/1(dout) -> t2/64
  correlator_i_instance1/2(vout) -> t3/1
  correlator_i_instance2/2(vout) -> t3/2
  correlator_i_instance3/2(vout) -> t3/3
  correlator_i_instance4/2(vout) -> t3/4
  correlator_i_instance5/2(vout) -> t3/5
  correlator_i_instance6/2(vout) -> t3/6
  correlator_i_instance7/2(vout) -> t3/7
  correlator_i_instance8/2(vout) -> t3/8
  correlator_i_instance9/2(vout) -> t3/9
  correlator_i_instance10/2(vout) -> t3/10
  correlator_i_instance11/2(vout) -> t3/11
  correlator_i_instance12/2(vout) -> t3/12
  correlator_i_instance13/2(vout) -> t3/13
  correlator_i_instance14/2(vout) -> t3/14
  correlator_i_instance15/2(vout) -> t3/15
  correlator_i_instance16/2(vout) -> t3/16
  correlator_i_instance17/2(vout) -> t3/17
  correlator_i_instance18/2(vout) -> t3/18
  correlator_i_instance19/2(vout) -> t3/19
  correlator_i_instance20/2(vout) -> t3/20
  correlator_i_instance21/2(vout) -> t3/21
  correlator_i_instance22/2(vout) -> t3/22
  correlator_i_instance23/2(vout) -> t3/23
  correlator_i_instance24/2(vout) -> t3/24
  correlator_i_instance25/2(vout) -> t3/25
  correlator_i_instance26/2(vout) -> t3/26
  correlator_i_instance27/2(vout) -> t3/27
  correlator_i_instance28/2(vout) -> t3/28
  correlator_i_instance29/2(vout) -> t3/29
  correlator_i_instance30/2(vout) -> t3/30
  correlator_i_instance31/2(vout) -> t3/31
  correlator_i_instance32/2(vout) -> t3/32
  correlator_i_instance33/2(vout) -> t3/33
  correlator_i_instance34/2(vout) -> t3/34
  correlator_i_instance35/2(vout) -> t3/35
  correlator_i_instance36/2(vout) -> t3/36
  correlator_i_instance37/2(vout) -> t3/37
  correlator_i_instance38/2(vout) -> t3/38
  correlator_i_instance39/2(vout) -> t3/39
  correlator_i_instance40/2(vout) -> t3/40
  correlator_i_instance41/2(vout) -> t3/41
  correlator_i_instance42/2(vout) -> t3/42
  correlator_i_instance43/2(vout) -> t3/43
  correlator_i_instance44/2(vout) -> t3/44
  correlator_i_instance45/2(vout) -> t3/45
  correlator_i_instance46/2(vout) -> t3/46
  correlator_i_instance47/2(vout) -> t3/47
  correlator_i_instance48/2(vout) -> t3/48
  correlator_i_instance49/2(vout) -> t3/49
  correlator_i_instance50/2(vout) -> t3/50
  correlator_i_instance51/2(vout) -> t3/51
  correlator_i_instance52/2(vout) -> t3/52
  correlator_i_instance53/2(vout) -> t3/53
  correlator_i_instance54/2(vout) -> t3/54
  correlator_i_instance55/2(vout) -> t3/55
  correlator_i_instance56/2(vout) -> t3/56
  correlator_i_instance57/2(vout) -> t3/57
  correlator_i_instance58/2(vout) -> t3/58
  correlator_i_instance59/2(vout) -> t3/59
  correlator_i_instance60/2(vout) -> t3/60
  correlator_i_instance61/2(vout) -> t3/61
  correlator_i_instance62/2(vout) -> t3/62
  correlator_i_instance63/2(vout) -> t3/63
  correlator_i_instance64/2(vout) -> t3/64
  t4/1 -> correlator_q_instance1/1(rx)
  t4/2 -> correlator_q_instance2/1(rx)
  t4/3 -> correlator_q_instance3/1(rx)
  t4/4 -> correlator_q_instance4/1(rx)
  t4/5 -> correlator_q_instance5/1(rx)
  t4/6 -> correlator_q_instance6/1(rx)
  t4/7 -> correlator_q_instance7/1(rx)
  t4/8 -> correlator_q_instance8/1(rx)
  t4/9 -> correlator_q_instance9/1(rx)
  t4/10 -> correlator_q_instance10/1(rx)
  t4/11 -> correlator_q_instance11/1(rx)
  t4/12 -> correlator_q_instance12/1(rx)
  t4/13 -> correlator_q_instance13/1(rx)
  t4/14 -> correlator_q_instance14/1(rx)
  t4/15 -> correlator_q_instance15/1(rx)
  t4/16 -> correlator_q_instance16/1(rx)
  t4/17 -> correlator_q_instance17/1(rx)
  t4/18 -> correlator_q_instance18/1(rx)
  t4/19 -> correlator_q_instance19/1(rx)
  t4/20 -> correlator_q_instance20/1(rx)
  t4/21 -> correlator_q_instance21/1(rx)
  t4/22 -> correlator_q_instance22/1(rx)
  t4/23 -> correlator_q_instance23/1(rx)
  t4/24 -> correlator_q_instance24/1(rx)
  t4/25 -> correlator_q_instance25/1(rx)
  t4/26 -> correlator_q_instance26/1(rx)
  t4/27 -> correlator_q_instance27/1(rx)
  t4/28 -> correlator_q_instance28/1(rx)
  t4/29 -> correlator_q_instance29/1(rx)
  t4/30 -> correlator_q_instance30/1(rx)
  t4/31 -> correlator_q_instance31/1(rx)
  t4/32 -> correlator_q_instance32/1(rx)
  t4/33 -> correlator_q_instance33/1(rx)
  t4/34 -> correlator_q_instance34/1(rx)
  t4/35 -> correlator_q_instance35/1(rx)
  t4/36 -> correlator_q_instance36/1(rx)
  t4/37 -> correlator_q_instance37/1(rx)
  t4/38 -> correlator_q_instance38/1(rx)
  t4/39 -> correlator_q_instance39/1(rx)
  t4/40 -> correlator_q_instance40/1(rx)
  t4/41 -> correlator_q_instance41/1(rx)
  t4/42 -> correlator_q_instance42/1(rx)
  t4/43 -> correlator_q_instance43/1(rx)
  t4/44 -> correlator_q_instance44/1(rx)
  t4/45 -> correlator_q_instance45/1(rx)
  t4/46 -> correlator_q_instance46/1(rx)
  t4/47 -> correlator_q_instance47/1(rx)
  t4/48 -> correlator_q_instance48/1(rx)
  t4/49 -> correlator_q_instance49/1(rx)
  t4/50 -> correlator_q_instance50/1(rx)
  t4/51 -> correlator_q_instance51/1(rx)
  t4/52 -> correlator_q_instance52/1(rx)
  t4/53 -> correlator_q_instance53/1(rx)
  t4/54 -> correlator_q_instance54/1(rx)
  t4/55 -> correlator_q_instance55/1(rx)
  t4/56 -> correlator_q_instance56/1(rx)
  t4/57 -> correlator_q_instance57/1(rx)
  t4/58 -> correlator_q_instance58/1(rx)
  t4/59 -> correlator_q_instance59/1(rx)
  t4/60 -> correlator_q_instance60/1(rx)
  t4/61 -> correlator_q_instance61/1(rx)
  t4/62 -> correlator_q_instance62/1(rx)
  t4/63 -> correlator_q_instance63/1(rx)
  t4/64 -> correlator_q_instance64/1(rx)
  t5/1 -> correlator_q_instance1/2(gs)
  t5/2 -> correlator_q_instance2/2(gs)
  t5/3 -> correlator_q_instance3/2(gs)
  t5/4 -> correlator_q_instance4/2(gs)
  t5/5 -> correlator_q_instance5/2(gs)
  t5/6 -> correlator_q_instance6/2(gs)
  t5/7 -> correlator_q_instance7/2(gs)
  t5/8 -> correlator_q_instance8/2(gs)
  t5/9 -> correlator_q_instance9/2(gs)
  t5/10 -> correlator_q_instance10/2(gs)
  t5/11 -> correlator_q_instance11/2(gs)
  t5/12 -> correlator_q_instance12/2(gs)
  t5/13 -> correlator_q_instance13/2(gs)
  t5/14 -> correlator_q_instance14/2(gs)
  t5/15 -> correlator_q_instance15/2(gs)
  t5/16 -> correlator_q_instance16/2(gs)
  t5/17 -> correlator_q_instance17/2(gs)
  t5/18 -> correlator_q_instance18/2(gs)
  t5/19 -> correlator_q_instance19/2(gs)
  t5/20 -> correlator_q_instance20/2(gs)
  t5/21 -> correlator_q_instance21/2(gs)
  t5/22 -> correlator_q_instance22/2(gs)
  t5/23 -> correlator_q_instance23/2(gs)
  t5/24 -> correlator_q_instance24/2(gs)
  t5/25 -> correlator_q_instance25/2(gs)
  t5/26 -> correlator_q_instance26/2(gs)
  t5/27 -> correlator_q_instance27/2(gs)
  t5/28 -> correlator_q_instance28/2(gs)
  t5/29 -> correlator_q_instance29/2(gs)
  t5/30 -> correlator_q_instance30/2(gs)
  t5/31 -> correlator_q_instance31/2(gs)
  t5/32 -> correlator_q_instance32/2(gs)
  t5/33 -> correlator_q_instance33/2(gs)
  t5/34 -> correlator_q_instance34/2(gs)
  t5/35 -> correlator_q_instance35/2(gs)
  t5/36 -> correlator_q_instance36/2(gs)
  t5/37 -> correlator_q_instance37/2(gs)
  t5/38 -> correlator_q_instance38/2(gs)
  t5/39 -> correlator_q_instance39/2(gs)
  t5/40 -> correlator_q_instance40/2(gs)
  t5/41 -> correlator_q_instance41/2(gs)
  t5/42 -> correlator_q_instance42/2(gs)
  t5/43 -> correlator_q_instance43/2(gs)
  t5/44 -> correlator_q_instance44/2(gs)
  t5/45 -> correlator_q_instance45/2(gs)
  t5/46 -> correlator_q_instance46/2(gs)
  t5/47 -> correlator_q_instance47/2(gs)
  t5/48 -> correlator_q_instance48/2(gs)
  t5/49 -> correlator_q_instance49/2(gs)
  t5/50 -> correlator_q_instance50/2(gs)
  t5/51 -> correlator_q_instance51/2(gs)
  t5/52 -> correlator_q_instance52/2(gs)
  t5/53 -> correlator_q_instance53/2(gs)
  t5/54 -> correlator_q_instance54/2(gs)
  t5/55 -> correlator_q_instance55/2(gs)
  t5/56 -> correlator_q_instance56/2(gs)
  t5/57 -> correlator_q_instance57/2(gs)
  t5/58 -> correlator_q_instance58/2(gs)
  t5/59 -> correlator_q_instance59/2(gs)
  t5/60 -> correlator_q_instance60/2(gs)
  t5/61 -> correlator_q_instance61/2(gs)
  t5/62 -> correlator_q_instance62/2(gs)
  t5/63 -> correlator_q_instance63/2(gs)
  t5/64 -> correlator_q_instance64/2(gs)
  correlator_q_instance1/1(dout) -> t6/1
  correlator_q_instance2/1(dout) -> t6/2
  correlator_q_instance3/1(dout) -> t6/3
  correlator_q_instance4/1(dout) -> t6/4
  correlator_q_instance5/1(dout) -> t6/5
  correlator_q_instance6/1(dout) -> t6/6
  correlator_q_instance7/1(dout) -> t6/7
  correlator_q_instance8/1(dout) -> t6/8
  correlator_q_instance9/1(dout) -> t6/9
  correlator_q_instance10/1(dout) -> t6/10
  correlator_q_instance11/1(dout) -> t6/11
  correlator_q_instance12/1(dout) -> t6/12
  correlator_q_instance13/1(dout) -> t6/13
  correlator_q_instance14/1(dout) -> t6/14
  correlator_q_instance15/1(dout) -> t6/15
  correlator_q_instance16/1(dout) -> t6/16
  correlator_q_instance17/1(dout) -> t6/17
  correlator_q_instance18/1(dout) -> t6/18
  correlator_q_instance19/1(dout) -> t6/19
  correlator_q_instance20/1(dout) -> t6/20
  correlator_q_instance21/1(dout) -> t6/21
  correlator_q_instance22/1(dout) -> t6/22
  correlator_q_instance23/1(dout) -> t6/23
  correlator_q_instance24/1(dout) -> t6/24
  correlator_q_instance25/1(dout) -> t6/25
  correlator_q_instance26/1(dout) -> t6/26
  correlator_q_instance27/1(dout) -> t6/27
  correlator_q_instance28/1(dout) -> t6/28
  correlator_q_instance29/1(dout) -> t6/29
  correlator_q_instance30/1(dout) -> t6/30
  correlator_q_instance31/1(dout) -> t6/31
  correlator_q_instance32/1(dout) -> t6/32
  correlator_q_instance33/1(dout) -> t6/33
  correlator_q_instance34/1(dout) -> t6/34
  correlator_q_instance35/1(dout) -> t6/35
  correlator_q_instance36/1(dout) -> t6/36
  correlator_q_instance37/1(dout) -> t6/37
  correlator_q_instance38/1(dout) -> t6/38
  correlator_q_instance39/1(dout) -> t6/39
  correlator_q_instance40/1(dout) -> t6/40
  correlator_q_instance41/1(dout) -> t6/41
  correlator_q_instance42/1(dout) -> t6/42
  correlator_q_instance43/1(dout) -> t6/43
  correlator_q_instance44/1(dout) -> t6/44
  correlator_q_instance45/1(dout) -> t6/45
  correlator_q_instance46/1(dout) -> t6/46
  correlator_q_instance47/1(dout) -> t6/47
  correlator_q_instance48/1(dout) -> t6/48
  correlator_q_instance49/1(dout) -> t6/49
  correlator_q_instance50/1(dout) -> t6/50
  correlator_q_instance51/1(dout) -> t6/51
  correlator_q_instance52/1(dout) -> t6/52
  correlator_q_instance53/1(dout) -> t6/53
  correlator_q_instance54/1(dout) -> t6/54
  correlator_q_instance55/1(dout) -> t6/55
  correlator_q_instance56/1(dout) -> t6/56
  correlator_q_instance57/1(dout) -> t6/57
  correlator_q_instance58/1(dout) -> t6/58
  correlator_q_instance59/1(dout) -> t6/59
  correlator_q_instance60/1(dout) -> t6/60
  correlator_q_instance61/1(dout) -> t6/61
  correlator_q_instance62/1(dout) -> t6/62
  correlator_q_instance63/1(dout) -> t6/63
  correlator_q_instance64/1(dout) -> t6/64
  correlator_q_instance1/2(vout) -> t7/1
  correlator_q_instance2/2(vout) -> t7/2
  correlator_q_instance3/2(vout) -> t7/3
  correlator_q_instance4/2(vout) -> t7/4
  correlator_q_instance5/2(vout) -> t7/5
  correlator_q_instance6/2(vout) -> t7/6
  correlator_q_instance7/2(vout) -> t7/7
  correlator_q_instance8/2(vout) -> t7/8
  correlator_q_instance9/2(vout) -> t7/9
  correlator_q_instance10/2(vout) -> t7/10
  correlator_q_instance11/2(vout) -> t7/11
  correlator_q_instance12/2(vout) -> t7/12
  correlator_q_instance13/2(vout) -> t7/13
  correlator_q_instance14/2(vout) -> t7/14
  correlator_q_instance15/2(vout) -> t7/15
  correlator_q_instance16/2(vout) -> t7/16
  correlator_q_instance17/2(vout) -> t7/17
  correlator_q_instance18/2(vout) -> t7/18
  correlator_q_instance19/2(vout) -> t7/19
  correlator_q_instance20/2(vout) -> t7/20
  correlator_q_instance21/2(vout) -> t7/21
  correlator_q_instance22/2(vout) -> t7/22
  correlator_q_instance23/2(vout) -> t7/23
  correlator_q_instance24/2(vout) -> t7/24
  correlator_q_instance25/2(vout) -> t7/25
  correlator_q_instance26/2(vout) -> t7/26
  correlator_q_instance27/2(vout) -> t7/27
  correlator_q_instance28/2(vout) -> t7/28
  correlator_q_instance29/2(vout) -> t7/29
  correlator_q_instance30/2(vout) -> t7/30
  correlator_q_instance31/2(vout) -> t7/31
  correlator_q_instance32/2(vout) -> t7/32
  correlator_q_instance33/2(vout) -> t7/33
  correlator_q_instance34/2(vout) -> t7/34
  correlator_q_instance35/2(vout) -> t7/35
  correlator_q_instance36/2(vout) -> t7/36
  correlator_q_instance37/2(vout) -> t7/37
  correlator_q_instance38/2(vout) -> t7/38
  correlator_q_instance39/2(vout) -> t7/39
  correlator_q_instance40/2(vout) -> t7/40
  correlator_q_instance41/2(vout) -> t7/41
  correlator_q_instance42/2(vout) -> t7/42
  correlator_q_instance43/2(vout) -> t7/43
  correlator_q_instance44/2(vout) -> t7/44
  correlator_q_instance45/2(vout) -> t7/45
  correlator_q_instance46/2(vout) -> t7/46
  correlator_q_instance47/2(vout) -> t7/47
  correlator_q_instance48/2(vout) -> t7/48
  correlator_q_instance49/2(vout) -> t7/49
  correlator_q_instance50/2(vout) -> t7/50
  correlator_q_instance51/2(vout) -> t7/51
  correlator_q_instance52/2(vout) -> t7/52
  correlator_q_instance53/2(vout) -> t7/53
  correlator_q_instance54/2(vout) -> t7/54
  correlator_q_instance55/2(vout) -> t7/55
  correlator_q_instance56/2(vout) -> t7/56
  correlator_q_instance57/2(vout) -> t7/57
  correlator_q_instance58/2(vout) -> t7/58
  correlator_q_instance59/2(vout) -> t7/59
  correlator_q_instance60/2(vout) -> t7/60
  correlator_q_instance61/2(vout) -> t7/61
  correlator_q_instance62/2(vout) -> t7/62
  correlator_q_instance63/2(vout) -> t7/63
  correlator_q_instance64/2(vout) -> t7/64
  t8/1 -> rx_ram_i_instance1/1(i)
  t8/2 -> rx_ram_i_instance2/1(i)
  t8/3 -> rx_ram_i_instance3/1(i)
  t8/4 -> rx_ram_i_instance4/1(i)
  t8/5 -> rx_ram_i_instance5/1(i)
  t8/6 -> rx_ram_i_instance6/1(i)
  t8/7 -> rx_ram_i_instance7/1(i)
  t8/8 -> rx_ram_i_instance8/1(i)
  t8/9 -> rx_ram_i_instance9/1(i)
  t8/10 -> rx_ram_i_instance10/1(i)
  t8/11 -> rx_ram_i_instance11/1(i)
  t8/12 -> rx_ram_i_instance12/1(i)
  t8/13 -> rx_ram_i_instance13/1(i)
  t8/14 -> rx_ram_i_instance14/1(i)
  t8/15 -> rx_ram_i_instance15/1(i)
  t8/16 -> rx_ram_i_instance16/1(i)
  t8/17 -> rx_ram_i_instance17/1(i)
  t8/18 -> rx_ram_i_instance18/1(i)
  t8/19 -> rx_ram_i_instance19/1(i)
  t8/20 -> rx_ram_i_instance20/1(i)
  t8/21 -> rx_ram_i_instance21/1(i)
  t8/22 -> rx_ram_i_instance22/1(i)
  t8/23 -> rx_ram_i_instance23/1(i)
  t8/24 -> rx_ram_i_instance24/1(i)
  t8/25 -> rx_ram_i_instance25/1(i)
  t8/26 -> rx_ram_i_instance26/1(i)
  t8/27 -> rx_ram_i_instance27/1(i)
  t8/28 -> rx_ram_i_instance28/1(i)
  t8/29 -> rx_ram_i_instance29/1(i)
  t8/30 -> rx_ram_i_instance30/1(i)
  t8/31 -> rx_ram_i_instance31/1(i)
  t8/32 -> rx_ram_i_instance32/1(i)
  t8/33 -> rx_ram_i_instance33/1(i)
  t8/34 -> rx_ram_i_instance34/1(i)
  t8/35 -> rx_ram_i_instance35/1(i)
  t8/36 -> rx_ram_i_instance36/1(i)
  t8/37 -> rx_ram_i_instance37/1(i)
  t8/38 -> rx_ram_i_instance38/1(i)
  t8/39 -> rx_ram_i_instance39/1(i)
  t8/40 -> rx_ram_i_instance40/1(i)
  t8/41 -> rx_ram_i_instance41/1(i)
  t8/42 -> rx_ram_i_instance42/1(i)
  t8/43 -> rx_ram_i_instance43/1(i)
  t8/44 -> rx_ram_i_instance44/1(i)
  t8/45 -> rx_ram_i_instance45/1(i)
  t8/46 -> rx_ram_i_instance46/1(i)
  t8/47 -> rx_ram_i_instance47/1(i)
  t8/48 -> rx_ram_i_instance48/1(i)
  t8/49 -> rx_ram_i_instance49/1(i)
  t8/50 -> rx_ram_i_instance50/1(i)
  t8/51 -> rx_ram_i_instance51/1(i)
  t8/52 -> rx_ram_i_instance52/1(i)
  t8/53 -> rx_ram_i_instance53/1(i)
  t8/54 -> rx_ram_i_instance54/1(i)
  t8/55 -> rx_ram_i_instance55/1(i)
  t8/56 -> rx_ram_i_instance56/1(i)
  t8/57 -> rx_ram_i_instance57/1(i)
  t8/58 -> rx_ram_i_instance58/1(i)
  t8/59 -> rx_ram_i_instance59/1(i)
  t8/60 -> rx_ram_i_instance60/1(i)
  t8/61 -> rx_ram_i_instance61/1(i)
  t8/62 -> rx_ram_i_instance62/1(i)
  t8/63 -> rx_ram_i_instance63/1(i)
  t8/64 -> rx_ram_i_instance64/1(i)
  rx_ram_i_instance1/1(dout) -> t9/1
  rx_ram_i_instance2/1(dout) -> t9/2
  rx_ram_i_instance3/1(dout) -> t9/3
  rx_ram_i_instance4/1(dout) -> t9/4
  rx_ram_i_instance5/1(dout) -> t9/5
  rx_ram_i_instance6/1(dout) -> t9/6
  rx_ram_i_instance7/1(dout) -> t9/7
  rx_ram_i_instance8/1(dout) -> t9/8
  rx_ram_i_instance9/1(dout) -> t9/9
  rx_ram_i_instance10/1(dout) -> t9/10
  rx_ram_i_instance11/1(dout) -> t9/11
  rx_ram_i_instance12/1(dout) -> t9/12
  rx_ram_i_instance13/1(dout) -> t9/13
  rx_ram_i_instance14/1(dout) -> t9/14
  rx_ram_i_instance15/1(dout) -> t9/15
  rx_ram_i_instance16/1(dout) -> t9/16
  rx_ram_i_instance17/1(dout) -> t9/17
  rx_ram_i_instance18/1(dout) -> t9/18
  rx_ram_i_instance19/1(dout) -> t9/19
  rx_ram_i_instance20/1(dout) -> t9/20
  rx_ram_i_instance21/1(dout) -> t9/21
  rx_ram_i_instance22/1(dout) -> t9/22
  rx_ram_i_instance23/1(dout) -> t9/23
  rx_ram_i_instance24/1(dout) -> t9/24
  rx_ram_i_instance25/1(dout) -> t9/25
  rx_ram_i_instance26/1(dout) -> t9/26
  rx_ram_i_instance27/1(dout) -> t9/27
  rx_ram_i_instance28/1(dout) -> t9/28
  rx_ram_i_instance29/1(dout) -> t9/29
  rx_ram_i_instance30/1(dout) -> t9/30
  rx_ram_i_instance31/1(dout) -> t9/31
  rx_ram_i_instance32/1(dout) -> t9/32
  rx_ram_i_instance33/1(dout) -> t9/33
  rx_ram_i_instance34/1(dout) -> t9/34
  rx_ram_i_instance35/1(dout) -> t9/35
  rx_ram_i_instance36/1(dout) -> t9/36
  rx_ram_i_instance37/1(dout) -> t9/37
  rx_ram_i_instance38/1(dout) -> t9/38
  rx_ram_i_instance39/1(dout) -> t9/39
  rx_ram_i_instance40/1(dout) -> t9/40
  rx_ram_i_instance41/1(dout) -> t9/41
  rx_ram_i_instance42/1(dout) -> t9/42
  rx_ram_i_instance43/1(dout) -> t9/43
  rx_ram_i_instance44/1(dout) -> t9/44
  rx_ram_i_instance45/1(dout) -> t9/45
  rx_ram_i_instance46/1(dout) -> t9/46
  rx_ram_i_instance47/1(dout) -> t9/47
  rx_ram_i_instance48/1(dout) -> t9/48
  rx_ram_i_instance49/1(dout) -> t9/49
  rx_ram_i_instance50/1(dout) -> t9/50
  rx_ram_i_instance51/1(dout) -> t9/51
  rx_ram_i_instance52/1(dout) -> t9/52
  rx_ram_i_instance53/1(dout) -> t9/53
  rx_ram_i_instance54/1(dout) -> t9/54
  rx_ram_i_instance55/1(dout) -> t9/55
  rx_ram_i_instance56/1(dout) -> t9/56
  rx_ram_i_instance57/1(dout) -> t9/57
  rx_ram_i_instance58/1(dout) -> t9/58
  rx_ram_i_instance59/1(dout) -> t9/59
  rx_ram_i_instance60/1(dout) -> t9/60
  rx_ram_i_instance61/1(dout) -> t9/61
  rx_ram_i_instance62/1(dout) -> t9/62
  rx_ram_i_instance63/1(dout) -> t9/63
  rx_ram_i_instance64/1(dout) -> t9/64
  t10/1 -> rx_ram_q_instance1/1(i)
  t10/2 -> rx_ram_q_instance2/1(i)
  t10/3 -> rx_ram_q_instance3/1(i)
  t10/4 -> rx_ram_q_instance4/1(i)
  t10/5 -> rx_ram_q_instance5/1(i)
  t10/6 -> rx_ram_q_instance6/1(i)
  t10/7 -> rx_ram_q_instance7/1(i)
  t10/8 -> rx_ram_q_instance8/1(i)
  t10/9 -> rx_ram_q_instance9/1(i)
  t10/10 -> rx_ram_q_instance10/1(i)
  t10/11 -> rx_ram_q_instance11/1(i)
  t10/12 -> rx_ram_q_instance12/1(i)
  t10/13 -> rx_ram_q_instance13/1(i)
  t10/14 -> rx_ram_q_instance14/1(i)
  t10/15 -> rx_ram_q_instance15/1(i)
  t10/16 -> rx_ram_q_instance16/1(i)
  t10/17 -> rx_ram_q_instance17/1(i)
  t10/18 -> rx_ram_q_instance18/1(i)
  t10/19 -> rx_ram_q_instance19/1(i)
  t10/20 -> rx_ram_q_instance20/1(i)
  t10/21 -> rx_ram_q_instance21/1(i)
  t10/22 -> rx_ram_q_instance22/1(i)
  t10/23 -> rx_ram_q_instance23/1(i)
  t10/24 -> rx_ram_q_instance24/1(i)
  t10/25 -> rx_ram_q_instance25/1(i)
  t10/26 -> rx_ram_q_instance26/1(i)
  t10/27 -> rx_ram_q_instance27/1(i)
  t10/28 -> rx_ram_q_instance28/1(i)
  t10/29 -> rx_ram_q_instance29/1(i)
  t10/30 -> rx_ram_q_instance30/1(i)
  t10/31 -> rx_ram_q_instance31/1(i)
  t10/32 -> rx_ram_q_instance32/1(i)
  t10/33 -> rx_ram_q_instance33/1(i)
  t10/34 -> rx_ram_q_instance34/1(i)
  t10/35 -> rx_ram_q_instance35/1(i)
  t10/36 -> rx_ram_q_instance36/1(i)
  t10/37 -> rx_ram_q_instance37/1(i)
  t10/38 -> rx_ram_q_instance38/1(i)
  t10/39 -> rx_ram_q_instance39/1(i)
  t10/40 -> rx_ram_q_instance40/1(i)
  t10/41 -> rx_ram_q_instance41/1(i)
  t10/42 -> rx_ram_q_instance42/1(i)
  t10/43 -> rx_ram_q_instance43/1(i)
  t10/44 -> rx_ram_q_instance44/1(i)
  t10/45 -> rx_ram_q_instance45/1(i)
  t10/46 -> rx_ram_q_instance46/1(i)
  t10/47 -> rx_ram_q_instance47/1(i)
  t10/48 -> rx_ram_q_instance48/1(i)
  t10/49 -> rx_ram_q_instance49/1(i)
  t10/50 -> rx_ram_q_instance50/1(i)
  t10/51 -> rx_ram_q_instance51/1(i)
  t10/52 -> rx_ram_q_instance52/1(i)
  t10/53 -> rx_ram_q_instance53/1(i)
  t10/54 -> rx_ram_q_instance54/1(i)
  t10/55 -> rx_ram_q_instance55/1(i)
  t10/56 -> rx_ram_q_instance56/1(i)
  t10/57 -> rx_ram_q_instance57/1(i)
  t10/58 -> rx_ram_q_instance58/1(i)
  t10/59 -> rx_ram_q_instance59/1(i)
  t10/60 -> rx_ram_q_instance60/1(i)
  t10/61 -> rx_ram_q_instance61/1(i)
  t10/62 -> rx_ram_q_instance62/1(i)
  t10/63 -> rx_ram_q_instance63/1(i)
  t10/64 -> rx_ram_q_instance64/1(i)
  rx_ram_q_instance1/1(dout) -> t11/1
  rx_ram_q_instance2/1(dout) -> t11/2
  rx_ram_q_instance3/1(dout) -> t11/3
  rx_ram_q_instance4/1(dout) -> t11/4
  rx_ram_q_instance5/1(dout) -> t11/5
  rx_ram_q_instance6/1(dout) -> t11/6
  rx_ram_q_instance7/1(dout) -> t11/7
  rx_ram_q_instance8/1(dout) -> t11/8
  rx_ram_q_instance9/1(dout) -> t11/9
  rx_ram_q_instance10/1(dout) -> t11/10
  rx_ram_q_instance11/1(dout) -> t11/11
  rx_ram_q_instance12/1(dout) -> t11/12
  rx_ram_q_instance13/1(dout) -> t11/13
  rx_ram_q_instance14/1(dout) -> t11/14
  rx_ram_q_instance15/1(dout) -> t11/15
  rx_ram_q_instance16/1(dout) -> t11/16
  rx_ram_q_instance17/1(dout) -> t11/17
  rx_ram_q_instance18/1(dout) -> t11/18
  rx_ram_q_instance19/1(dout) -> t11/19
  rx_ram_q_instance20/1(dout) -> t11/20
  rx_ram_q_instance21/1(dout) -> t11/21
  rx_ram_q_instance22/1(dout) -> t11/22
  rx_ram_q_instance23/1(dout) -> t11/23
  rx_ram_q_instance24/1(dout) -> t11/24
  rx_ram_q_instance25/1(dout) -> t11/25
  rx_ram_q_instance26/1(dout) -> t11/26
  rx_ram_q_instance27/1(dout) -> t11/27
  rx_ram_q_instance28/1(dout) -> t11/28
  rx_ram_q_instance29/1(dout) -> t11/29
  rx_ram_q_instance30/1(dout) -> t11/30
  rx_ram_q_instance31/1(dout) -> t11/31
  rx_ram_q_instance32/1(dout) -> t11/32
  rx_ram_q_instance33/1(dout) -> t11/33
  rx_ram_q_instance34/1(dout) -> t11/34
  rx_ram_q_instance35/1(dout) -> t11/35
  rx_ram_q_instance36/1(dout) -> t11/36
  rx_ram_q_instance37/1(dout) -> t11/37
  rx_ram_q_instance38/1(dout) -> t11/38
  rx_ram_q_instance39/1(dout) -> t11/39
  rx_ram_q_instance40/1(dout) -> t11/40
  rx_ram_q_instance41/1(dout) -> t11/41
  rx_ram_q_instance42/1(dout) -> t11/42
  rx_ram_q_instance43/1(dout) -> t11/43
  rx_ram_q_instance44/1(dout) -> t11/44
  rx_ram_q_instance45/1(dout) -> t11/45
  rx_ram_q_instance46/1(dout) -> t11/46
  rx_ram_q_instance47/1(dout) -> t11/47
  rx_ram_q_instance48/1(dout) -> t11/48
  rx_ram_q_instance49/1(dout) -> t11/49
  rx_ram_q_instance50/1(dout) -> t11/50
  rx_ram_q_instance51/1(dout) -> t11/51
  rx_ram_q_instance52/1(dout) -> t11/52
  rx_ram_q_instance53/1(dout) -> t11/53
  rx_ram_q_instance54/1(dout) -> t11/54
  rx_ram_q_instance55/1(dout) -> t11/55
  rx_ram_q_instance56/1(dout) -> t11/56
  rx_ram_q_instance57/1(dout) -> t11/57
  rx_ram_q_instance58/1(dout) -> t11/58
  rx_ram_q_instance59/1(dout) -> t11/59
  rx_ram_q_instance60/1(dout) -> t11/60
  rx_ram_q_instance61/1(dout) -> t11/61
  rx_ram_q_instance62/1(dout) -> t11/62
  rx_ram_q_instance63/1(dout) -> t11/63
  rx_ram_q_instance64/1(dout) -> t11/64
  t12/1 -> sum_elements_i_instance1/1(din)
  t12/2 -> sum_elements_i_instance2/1(din)
  t12/3 -> sum_elements_i_instance3/1(din)
  t12/4 -> sum_elements_i_instance4/1(din)
  t12/5 -> sum_elements_i_instance5/1(din)
  t12/6 -> sum_elements_i_instance6/1(din)
  t12/7 -> sum_elements_i_instance7/1(din)
  t12/8 -> sum_elements_i_instance8/1(din)
  sum_elements_i_instance1/1(dout) -> t13/1
  sum_elements_i_instance2/1(dout) -> t13/2
  sum_elements_i_instance3/1(dout) -> t13/3
  sum_elements_i_instance4/1(dout) -> t13/4
  sum_elements_i_instance5/1(dout) -> t13/5
  sum_elements_i_instance6/1(dout) -> t13/6
  sum_elements_i_instance7/1(dout) -> t13/7
  sum_elements_i_instance8/1(dout) -> t13/8
  sum_elements_i_instance1/2(vout) -> t14/1
  sum_elements_i_instance2/2(vout) -> t14/2
  sum_elements_i_instance3/2(vout) -> t14/3
  sum_elements_i_instance4/2(vout) -> t14/4
  sum_elements_i_instance5/2(vout) -> t14/5
  sum_elements_i_instance6/2(vout) -> t14/6
  sum_elements_i_instance7/2(vout) -> t14/7
  sum_elements_i_instance8/2(vout) -> t14/8
  t15/1 -> sum_elements_q_instance1/1(din)
  t15/2 -> sum_elements_q_instance2/1(din)
  t15/3 -> sum_elements_q_instance3/1(din)
  t15/4 -> sum_elements_q_instance4/1(din)
  t15/5 -> sum_elements_q_instance5/1(din)
  t15/6 -> sum_elements_q_instance6/1(din)
  t15/7 -> sum_elements_q_instance7/1(din)
  t15/8 -> sum_elements_q_instance8/1(din)
  sum_elements_q_instance1/1(dout) -> t16/1
  sum_elements_q_instance2/1(dout) -> t16/2
  sum_elements_q_instance3/1(dout) -> t16/3
  sum_elements_q_instance4/1(dout) -> t16/4
  sum_elements_q_instance5/1(dout) -> t16/5
  sum_elements_q_instance6/1(dout) -> t16/6
  sum_elements_q_instance7/1(dout) -> t16/7
  sum_elements_q_instance8/1(dout) -> t16/8
  sum_elements_q_instance1/2(vout) -> t17/1
  sum_elements_q_instance2/2(vout) -> t17/2
  sum_elements_q_instance3/2(vout) -> t17/3
  sum_elements_q_instance4/2(vout) -> t17/4
  sum_elements_q_instance5/2(vout) -> t17/5
  sum_elements_q_instance6/2(vout) -> t17/6
  sum_elements_q_instance7/2(vout) -> t17/7
  sum_elements_q_instance8/2(vout) -> t17/8
